simulink model "hcu_main_ADASwEPS"  (Simulink 8.2)
settings: Solver=FixedStepDiscrete  StartTime=0.0  StopTime=inf  FixedStep=0.001  RelTol=1e-3
PostLoadFcn:
  | , if any(exist('dsrtsu_mdlpostloadfcn', 'file') == [2, 3, 6]), try dsrtsu_mdlpostloadfcn('Execute', bdroot); catch fprintf('Error in PostLoadFcn (dsrtsu_mdlpostloadfcn) for model "%s":\n %s\n', bdroot, lasterr); end, end,
values from neighbouring files (symbols this model uses):
  C_TASK_1MS_S = (	C_TICK_TIME_S       )    [hcu_local_hdr.m]    (also in temp_ovrd_values.m = double(	0.001                  ))
  C_TICK_TIME_S = single(	0.005	    	)    [hcu_local_hdr.m]
  ENUM_EPSLFCSTATUS_ACTIVE = uint8(  2  )    [hcu_local_hdr.m]
  ENUM_EPSLFCSTATUS_TRANSITION = uint8(  3  )    [hcu_local_hdr.m]
  ENUM_EPSLKASTATUS_ACTIVE = uint8(  2  )    [hcu_local_hdr.m]
  ENUM_EPSMODEREQ_ANGLE = uint8(  1  )    [hcu_local_hdr.m]
  ENUM_EPSMODEREQ_INTERNAL = uint8(  0  )    [hcu_local_hdr.m]
  ENUM_EPSMODEREQ_TORQUE = uint8(  2  )    [hcu_local_hdr.m]
  ENUM_GEARPOSN_1ST = uint8(  1  )    [hcu_local_hdr.m]
  ENUM_GEARPOSN_2ND = uint8(  2  )    [hcu_local_hdr.m]
  ENUM_GEARPOSN_3RD = uint8(  3  )    [hcu_local_hdr.m]
  ENUM_GEARPOSN_4TH = uint8(  4  )    [hcu_local_hdr.m]
  ENUM_GEARPOSN_5TH = uint8(  5  )    [hcu_local_hdr.m]
  ENUM_GEARPOSN_6TH = uint8(  6  )    [hcu_local_hdr.m]
  ENUM_GEARPOSN_R = uint8(  7  )    [hcu_local_hdr.m]
  FALSE = boolean( 0 )    [hcu_local_hdr.m]
  TRUE = boolean( 1 )    [hcu_local_hdr.m]
undefined symbols (not defined in the file or in its folder): AISP_EPSCurrent_pct, AISP_TqASensorDelta_pct, AISP_TqBSensorDelta_pct, dHAL_IN, hal, INVALID_ABS1_TIMEOUT, INVALID_ABS2_TIMEOUT, INVALID_ABS3_TIMEOUT, INVALID_ABS4_TIMEOUT, INVALID_AC1_TIMEOUT, INVALID_ADASTORQ_REQ, INVALID_BCM1_TIMEOUT, INVALID_BCM2_TIMEOUT, INVALID_BOOSTER_VAC, INVALID_CSW1_TIMEOUT, INVALID_CUR_VEHDECE, INVALID_CURBRAKEDECE_REQ, INVALID_CURSTEERANG_REQ, INVALID_CURSTEERTQ_REQ, INVALID_ECM1_TIMEOUT, INVALID_ECM2_TIMEOUT, INVALID_ECM3_TIMEOUT, INVALID_ECM9_TIMEOUT, INVALID_ENG_TORQUE_FRICTIONAL, INVALID_ENG_TORQUE_INDICATED, INVALID_ENG_TORQUE_INDICATEDCOR, INVALID_ENG_TQ_MAX, INVALID_ENG_TQ_MIN, INVALID_EPAS2_TIMEOUT, INVALID_EPAS3_TIMEOUT, INVALID_EPB1_TIMEOUT, INVALID_EPS_BATTVOLT, INVALID_ESC_BATTVOLT, INVALID_GRADE, INVALID_HCU3_TIMEOUT, INVALID_HCU4_TIMEOUT, INVALID_HMI1_TIMEOUT, INVALID_HMI2_TIMEOUT, INVALID_LAT_ACC, INVALID_LONG_ACC, INVALID_MC_PRESSURE, INVALID_METER1_TIMEOUT, INVALID_METER3_TIMEOUT, INVALID_METER_VEHSPD, INVALID_ODO_METER, INVALID_OUTSIDE_TEMP, INVALID_PARKBRAKEBIND_STAT, INVALID_PEDALTQ_REQ, INVALID_SAS1_TIMEOUT, INVALID_SAS_ANGLE, INVALID_SHIFTER_POSN, INVALID_TCM1_TIMEOUT, INVALID_TCM2_TIMEOUT, INVALID_VCU1_TIMEOUT, INVALID_VCU2_TIMEOUT, INVALID_VEH_CRASH, INVALID_VEH_SPD, INVALID_WHEEL_SPD, INVALID_YAW_RATE, KHAL_MssgIdObj1_num ... (+8)
libraries: simulink x147, hcu_lib x38, rti1401lib_dio_type3 x4, rtimmsu_dsrtlib x3, app x1, rtiethernetudplib x1, rti1401lib_adc_type4 x1, rti1401lib_dac_type3 x1, inp x1, lidr x1, outp x1
(part 7 of 15)

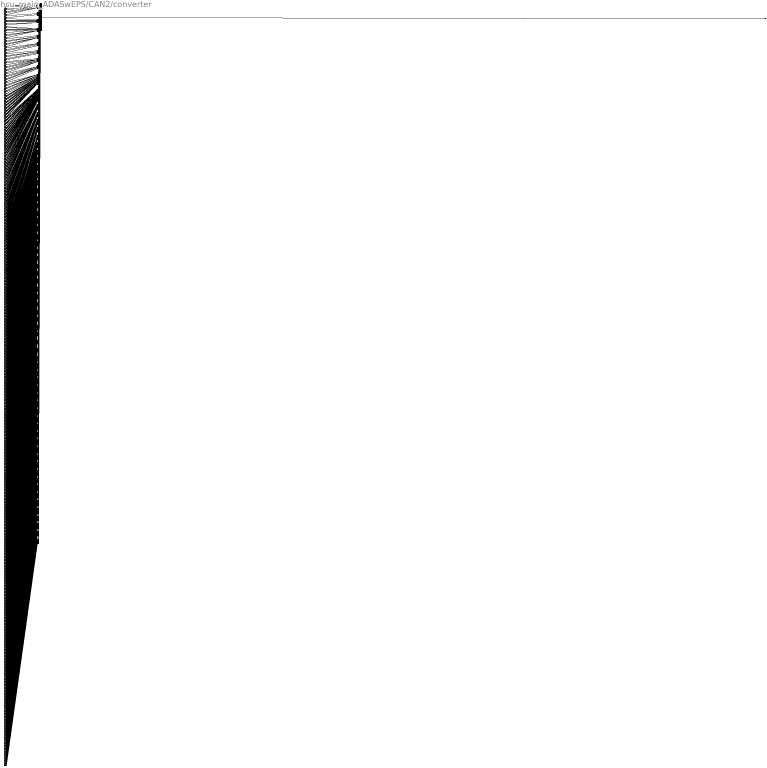
== system hcu_main_ADASwEPS/CAN2/converter ==
  in_1 : Inport
  in_2 : Inport  Port=2
  in_3 : Inport  Port=3
  in_4 : Inport  Port=4
  in_5 : Inport  Port=5
  in_6 : Inport  Port=6
  in_7 : Inport  Port=7
  in_8 : Inport  Port=8
  in_9 : Inport  Port=9
  in_10 : Inport  Port=10
  in_11 : Inport  Port=11
  in_12 : Inport  Port=12
  in_13 : Inport  Port=13
  in_14 : Inport  Port=14
  in_15 : Inport  Port=15
  in_16 : Inport  Port=16
  in_17 : Inport  Port=17
  in_18 : Inport  Port=18
  in_19 : Inport  Port=19
  in_20 : Inport  Port=20
  in_21 : Inport  Port=21
  in_22 : Inport  Port=22
  in_23 : Inport  Port=23
  in_24 : Inport  Port=24
  in_25 : Inport  Port=25
  in_26 : Inport  Port=26
  in_27 : Inport  Port=27
  in_28 : Inport  Port=28
  in_29 : Inport  Port=29
  in_30 : Inport  Port=30
  in_31 : Inport  Port=31
  in_32 : Inport  Port=32
  in_33 : Inport  Port=33
  in_34 : Inport  Port=34
  in_35 : Inport  Port=35
  in_36 : Inport  Port=36
  in_37 : Inport  Port=37
  in_38 : Inport  Port=38
  in_39 : Inport  Port=39
  in_40 : Inport  Port=40
  in_41 : Inport  Port=41
  in_42 : Inport  Port=42
  in_43 : Inport  Port=43
  in_44 : Inport  Port=44
  in_45 : Inport  Port=45
  in_46 : Inport  Port=46
  in_47 : Inport  Port=47
  in_48 : Inport  Port=48
  in_49 : Inport  Port=49
  in_50 : Inport  Port=50
  in_51 : Inport  Port=51
  in_52 : Inport  Port=52
  in_53 : Inport  Port=53
  in_54 : Inport  Port=54
  in_55 : Inport  Port=55
  in_56 : Inport  Port=56
  in_57 : Inport  Port=57
  in_58 : Inport  Port=58
  in_59 : Inport  Port=59
  in_60 : Inport  Port=60
  in_61 : Inport  Port=61
  in_62 : Inport  Port=62
  in_63 : Inport  Port=63
  in_64 : Inport  Port=64
  in_65 : Inport  Port=65
  in_66 : Inport  Port=66
  in_67 : Inport  Port=67
  in_68 : Inport  Port=68
  in_69 : Inport  Port=69
  in_70 : Inport  Port=70
  in_71 : Inport  Port=71
  in_72 : Inport  Port=72
  in_73 : Inport  Port=73
  in_74 : Inport  Port=74
  in_75 : Inport  Port=75
  in_76 : Inport  Port=76
  in_77 : Inport  Port=77
  in_78 : Inport  Port=78
  in_79 : Inport  Port=79
  in_80 : Inport  Port=80
  in_81 : Inport  Port=81
  in_82 : Inport  Port=82
  in_83 : Inport  Port=83
  in_84 : Inport  Port=84
  in_85 : Inport  Port=85
  in_86 : Inport  Port=86
  in_87 : Inport  Port=87
  in_88 : Inport  Port=88
  in_89 : Inport  Port=89
  in_90 : Inport  Port=90
  in_91 : Inport  Port=91
  in_92 : Inport  Port=92
  in_93 : Inport  Port=93
  in_94 : Inport  Port=94
  in_95 : Inport  Port=95
  in_96 : Inport  Port=96
  in_97 : Inport  Port=97
  in_98 : Inport  Port=98
  in_99 : Inport  Port=99
  in_100 : Inport  Port=100
  in_101 : Inport  Port=101
  in_102 : Inport  Port=102
  in_103 : Inport  Port=103
  in_104 : Inport  Port=104
  in_105 : Inport  Port=105
  in_106 : Inport  Port=106
  in_107 : Inport  Port=107
  in_108 : Inport  Port=108
  in_109 : Inport  Port=109
  in_110 : Inport  Port=110
  in_111 : Inport  Port=111
  in_112 : Inport  Port=112
  in_113 : Inport  Port=113
  in_114 : Inport  Port=114
  in_115 : Inport  Port=115
  in_116 : Inport  Port=116
  in_117 : Inport  Port=117
  in_118 : Inport  Port=118
  in_119 : Inport  Port=119
  in_120 : Inport  Port=120
  in_121 : Inport  Port=121
  in_122 : Inport  Port=122
  in_123 : Inport  Port=123
  in_124 : Inport  Port=124
  in_125 : Inport  Port=125
  in_126 : Inport  Port=126
  in_127 : Inport  Port=127
  in_128 : Inport  Port=128
  in_129 : Inport  Port=129
  in_130 : Inport  Port=130
  in_131 : Inport  Port=131
  in_132 : Inport  Port=132
  in_133 : Inport  Port=133
  in_134 : Inport  Port=134
  in_135 : Inport  Port=135
  in_136 : Inport  Port=136
  in_137 : Inport  Port=137
  in_138 : Inport  Port=138
  in_139 : Inport  Port=139
  in_140 : Inport  Port=140
  in_141 : Inport  Port=141
  in_142 : Inport  Port=142
  in_143 : Inport  Port=143
  in_144 : Inport  Port=144
  in_145 : Inport  Port=145
  in_146 : Inport  Port=146
  in_147 : Inport  Port=147
  in_148 : Inport  Port=148
  in_149 : Inport  Port=149
  in_150 : Inport  Port=150
  in_151 : Inport  Port=151
  in_152 : Inport  Port=152
  in_153 : Inport  Port=153
  in_154 : Inport  Port=154
  in_155 : Inport  Port=155
  in_156 : Inport  Port=156
  in_157 : Inport  Port=157
  in_158 : Inport  Port=158
  in_159 : Inport  Port=159
  in_160 : Inport  Port=160
  in_161 : Inport  Port=161
  in_162 : Inport  Port=162
  in_163 : Inport  Port=163
  in_164 : Inport  Port=164
  in_165 : Inport  Port=165
  in_166 : Inport  Port=166
  in_167 : Inport  Port=167
  in_168 : Inport  Port=168
  in_169 : Inport  Port=169
  in_170 : Inport  Port=170
  in_171 : Inport  Port=171
  in_172 : Inport  Port=172
  in_173 : Inport  Port=173
  in_174 : Inport  Port=174
  in_175 : Inport  Port=175
  in_176 : Inport  Port=176
  in_177 : Inport  Port=177
  in_178 : Inport  Port=178
  in_179 : Inport  Port=179
  in_180 : Inport  Port=180
  in_181 : Inport  Port=181
  in_182 : Inport  Port=182
  in_183 : Inport  Port=183
  in_184 : Inport  Port=184
  in_185 : Inport  Port=185
  in_186 : Inport  Port=186
  in_187 : Inport  Port=187
  in_188 : Inport  Port=188
  in_189 : Inport  Port=189
  in_190 : Inport  Port=190
  in_191 : Inport  Port=191
  in_192 : Inport  Port=192
  in_193 : Inport  Port=193
  in_194 : Inport  Port=194
  in_195 : Inport  Port=195
  in_196 : Inport  Port=196
  in_197 : Inport  Port=197
  in_198 : Inport  Port=198
  in_199 : Inport  Port=199
  in_200 : Inport  Port=200
  in_201 : Inport  Port=201
  in_202 : Inport  Port=202
  in_203 : Inport  Port=203
  in_204 : Inport  Port=204
  in_205 : Inport  Port=205
  in_206 : Inport  Port=206
  in_207 : Inport  Port=207
  in_208 : Inport  Port=208
  in_209 : Inport  Port=209
  in_210 : Inport  Port=210
  in_211 : Inport  Port=211
  in_212 : Inport  Port=212
  in_213 : Inport  Port=213
  in_214 : Inport  Port=214
  in_215 : Inport  Port=215
  in_216 : Inport  Port=216
  in_217 : Inport  Port=217
  in_218 : Inport  Port=218
  in_219 : Inport  Port=219
  in_220 : Inport  Port=220
  in_221 : Inport  Port=221
  in_222 : Inport  Port=222
  in_223 : Inport  Port=223
  in_224 : Inport  Port=224
  in_225 : Inport  Port=225
  in_226 : Inport  Port=226
  in_227 : Inport  Port=227
  in_228 : Inport  Port=228
  in_229 : Inport  Port=229
  in_230 : Inport  Port=230
  in_231 : Inport  Port=231
  in_232 : Inport  Port=232
  in_233 : Inport  Port=233
  in_234 : Inport  Port=234
  in_235 : Inport  Port=235
  in_236 : Inport  Port=236
  in_237 : Inport  Port=237
  in_238 : Inport  Port=238
  in_239 : Inport  Port=239
  in_240 : Inport  Port=240
  in_241 : Inport  Port=241
  in_242 : Inport  Port=242
  in_243 : Inport  Port=243
  in_244 : Inport  Port=244
  in_245 : Inport  Port=245
  in_246 : Inport  Port=246
  in_247 : Inport  Port=247
  in_248 : Inport  Port=248
  in_249 : Inport  Port=249
  in_250 : Inport  Port=250
  in_251 : Inport  Port=251
  in_252 : Inport  Port=252
  in_253 : Inport  Port=253
  in_254 : Inport  Port=254
  in_255 : Inport  Port=255
  in_256 : Inport  Port=256
  in_257 : Inport  Port=257
  in_258 : Inport  Port=258
  in_259 : Inport  Port=259
  in_260 : Inport  Port=260
  in_261 : Inport  Port=261
  in_262 : Inport  Port=262
  in_263 : Inport  Port=263
  in_264 : Inport  Port=264
  in_265 : Inport  Port=265
  in_266 : Inport  Port=266
  in_267 : Inport  Port=267
  in_268 : Inport  Port=268
  in_269 : Inport  Port=269
  in_270 : Inport  Port=270
  in_271 : Inport  Port=271
  in_272 : Inport  Port=272
  in_273 : Inport  Port=273
  in_274 : Inport  Port=274
  in_275 : Inport  Port=275
  in_276 : Inport  Port=276
  in_277 : Inport  Port=277
  in_278 : Inport  Port=278
  in_279 : Inport  Port=279
  in_280 : Inport  Port=280
  in_281 : Inport  Port=281
  in_282 : Inport  Port=282
  in_283 : Inport  Port=283
  in_284 : Inport  Port=284
  in_285 : Inport  Port=285
  in_286 : Inport  Port=286
  in_287 : Inport  Port=287
  in_288 : Inport  Port=288
  in_289 : Inport  Port=289
  in_290 : Inport  Port=290
  in_291 : Inport  Port=291
  in_292 : Inport  Port=292
  in_293 : Inport  Port=293
  in_294 : Inport  Port=294
  in_295 : Inport  Port=295
  in_296 : Inport  Port=296
  in_297 : Inport  Port=297
  in_298 : Inport  Port=298
  in_299 : Inport  Port=299
  in_300 : Inport  Port=300
  in_301 : Inport  Port=301
  in_302 : Inport  Port=302
  in_303 : Inport  Port=303
  in_304 : Inport  Port=304
  in_305 : Inport  Port=305
  in_306 : Inport  Port=306
  in_307 : Inport  Port=307
  in_308 : Inport  Port=308
  in_309 : Inport  Port=309
  in_310 : Inport  Port=310
  in_311 : Inport  Port=311
  in_312 : Inport  Port=312
  in_313 : Inport  Port=313
  in_314 : Inport  Port=314
  in_315 : Inport  Port=315
  in_316 : Inport  Port=316
  in_317 : Inport  Port=317
  in_318 : Inport  Port=318
  in_319 : Inport  Port=319
  in_320 : Inport  Port=320
  in_321 : Inport  Port=321
  in_322 : Inport  Port=322
  in_323 : Inport  Port=323
  in_324 : Inport  Port=324
  in_325 : Inport  Port=325
  in_326 : Inport  Port=326
  in_327 : Inport  Port=327
  in_328 : Inport  Port=328
  in_329 : Inport  Port=329
  in_330 : Inport  Port=330
  in_331 : Inport  Port=331
  in_332 : Inport  Port=332
  in_333 : Inport  Port=333
  in_334 : Inport  Port=334
  in_335 : Inport  Port=335
  in_336 : Inport  Port=336
  in_337 : Inport  Port=337
  in_338 : Inport  Port=338
  in_339 : Inport  Port=339
  in_340 : Inport  Port=340
  in_341 : Inport  Port=341
  in_342 : Inport  Port=342
  in_343 : Inport  Port=343
  in_344 : Inport  Port=344
  in_345 : Inport  Port=345
  in_346 : Inport  Port=346
  in_347 : Inport  Port=347
  in_348 : Inport  Port=348
  in_349 : Inport  Port=349
  in_350 : Inport  Port=350
  in_351 : Inport  Port=351
  in_352 : Inport  Port=352
  in_353 : Inport  Port=353
  in_354 : Inport  Port=354
  in_355 : Inport  Port=355
  in_356 : Inport  Port=356
  in_357 : Inport  Port=357
  in_358 : Inport  Port=358
  in_359 : Inport  Port=359
  in_360 : Inport  Port=360
  in_361 : Inport  Port=361
  in_362 : Inport  Port=362
  in_363 : Inport  Port=363
  in_364 : Inport  Port=364
  in_365 : Inport  Port=365
  in_366 : Inport  Port=366
  in_367 : Inport  Port=367
  in_368 : Inport  Port=368
  in_369 : Inport  Port=369
  in_370 : Inport  Port=370
  in_371 : Inport  Port=371
  in_372 : Inport  Port=372
  in_373 : Inport  Port=373
  in_374 : Inport  Port=374
  in_375 : Inport  Port=375
  in_376 : Inport  Port=376
  in_377 : Inport  Port=377
  in_378 : Inport  Port=378
  in_379 : Inport  Port=379
  in_380 : Inport  Port=380
  in_381 : Inport  Port=381
  in_382 : Inport  Port=382
  in_383 : Inport  Port=383
  in_384 : Inport  Port=384
  in_385 : Inport  Port=385
  in_386 : Inport  Port=386
  in_387 : Inport  Port=387
  in_388 : Inport  Port=388
  in_389 : Inport  Port=389
  in_390 : Inport  Port=390
  in_391 : Inport  Port=391
  in_392 : Inport  Port=392
  in_393 : Inport  Port=393
  in_394 : Inport  Port=394
  in_395 : Inport  Port=395
  in_396 : Inport  Port=396
  in_397 : Inport  Port=397
  in_398 : Inport  Port=398
  in_399 : Inport  Port=399
  in_400 : Inport  Port=400
  in_401 : Inport  Port=401
  in_402 : Inport  Port=402
  in_403 : Inport  Port=403
  in_404 : Inport  Port=404
  in_405 : Inport  Port=405
  in_406 : Inport  Port=406
  in_407 : Inport  Port=407
  in_408 : Inport  Port=408
  in_409 : Inport  Port=409
  in_410 : Inport  Port=410
  in_411 : Inport  Port=411
  in_412 : Inport  Port=412
  in_413 : Inport  Port=413
  in_414 : Inport  Port=414
  in_415 : Inport  Port=415
  in_416 : Inport  Port=416
  in_417 : Inport  Port=417
  in_418 : Inport  Port=418
  in_419 : Inport  Port=419
  in_420 : Inport  Port=420
  in_421 : Inport  Port=421
  in_422 : Inport  Port=422
  in_423 : Inport  Port=423
  in_424 : Inport  Port=424
  in_425 : Inport  Port=425
  in_426 : Inport  Port=426
  in_427 : Inport  Port=427
  in_428 : Inport  Port=428
  in_429 : Inport  Port=429
  in_430 : Inport  Port=430
  in_431 : Inport  Port=431
  in_432 : Inport  Port=432
  in_433 : Inport  Port=433
  in_434 : Inport  Port=434
  in_435 : Inport  Port=435
  in_436 : Inport  Port=436
  in_437 : Inport  Port=437
  in_438 : Inport  Port=438
  in_439 : Inport  Port=439
  in_440 : Inport  Port=440
  in_441 : Inport  Port=441
  in_442 : Inport  Port=442
  in_443 : Inport  Port=443
  in_444 : Inport  Port=444
  in_445 : Inport  Port=445
  in_446 : Inport  Port=446
  in_447 : Inport  Port=447
  in_448 : Inport  Port=448
  in_449 : Inport  Port=449
  in_450 : Inport  Port=450
  in_451 : Inport  Port=451
  in_452 : Inport  Port=452
  in_453 : Inport  Port=453
  in_454 : Inport  Port=454
  in_455 : Inport  Port=455
  in_456 : Inport  Port=456
  in_457 : Inport  Port=457
  in_458 : Inport  Port=458
  in_459 : Inport  Port=459
  in_460 : Inport  Port=460
  in_461 : Inport  Port=461
  in_462 : Inport  Port=462
  in_463 : Inport  Port=463
  in_464 : Inport  Port=464
  in_465 : Inport  Port=465
  in_466 : Inport  Port=466
  in_467 : Inport  Port=467
  in_468 : Inport  Port=468
  in_469 : Inport  Port=469
  in_470 : Inport  Port=470
  in_471 : Inport  Port=471
  in_472 : Inport  Port=472
  in_473 : Inport  Port=473
  in_474 : Inport  Port=474
  in_475 : Inport  Port=475
  in_476 : Inport  Port=476
  in_477 : Inport  Port=477
  in_478 : Inport  Port=478
  in_479 : Inport  Port=479
  in_480 : Inport  Port=480
  in_481 : Inport  Port=481
  in_482 : Inport  Port=482
  in_483 : Inport  Port=483
  in_484 : Inport  Port=484
  in_485 : Inport  Port=485
  in_486 : Inport  Port=486
  in_487 : Inport  Port=487
  in_488 : Inport  Port=488
  in_489 : Inport  Port=489
  in_490 : Inport  Port=490
  in_491 : Inport  Port=491
  in_492 : Inport  Port=492
  in_493 : Inport  Port=493
  in_494 : Inport  Port=494
  in_495 : Inport  Port=495
  in_496 : Inport  Port=496
  in_497 : Inport  Port=497
  in_498 : Inport  Port=498
  in_499 : Inport  Port=499
  in_500 : Inport  Port=500
  in_501 : Inport  Port=501
  in_502 : Inport  Port=502
  in_503 : Inport  Port=503
  in_504 : Inport  Port=504
  in_505 : Inport  Port=505
  in_506 : Inport  Port=506
  in_507 : Inport  Port=507
  in_508 : Inport  Port=508
  in_509 : Inport  Port=509
  in_510 : Inport  Port=510
  in_511 : Inport  Port=511
  in_512 : Inport  Port=512
  in_513 : Inport  Port=513
  in_514 : Inport  Port=514
  in_515 : Inport  Port=515
  in_516 : Inport  Port=516
  in_517 : Inport  Port=517
  in_518 : Inport  Port=518
  in_519 : Inport  Port=519
  in_520 : Inport  Port=520
  in_521 : Inport  Port=521
  in_522 : Inport  Port=522
  in_523 : Inport  Port=523
  in_524 : Inport  Port=524
  in_525 : Inport  Port=525
  in_526 : Inport  Port=526
  in_527 : Inport  Port=527
  in_528 : Inport  Port=528
  in_529 : Inport  Port=529
  in_530 : Inport  Port=530
  in_531 : Inport  Port=531
  in_532 : Inport  Port=532
  in_533 : Inport  Port=533
  in_534 : Inport  Port=534
  in_535 : Inport  Port=535
  in_536 : Inport  Port=536
  in_537 : Inport  Port=537
  in_538 : Inport  Port=538
  in_539 : Inport  Port=539
  in_540 : Inport  Port=540
  in_541 : Inport  Port=541
  in_542 : Inport  Port=542
  in_543 : Inport  Port=543
  in_544 : Inport  Port=544
  in_545 : Inport  Port=545
  in_546 : Inport  Port=546
  in_547 : Inport  Port=547
  in_548 : Inport  Port=548
  in_549 : Inport  Port=549
  in_550 : Inport  Port=550
  in_551 : Inport  Port=551
  in_552 : Inport  Port=552
  in_553 : Inport  Port=553
  in_554 : Inport  Port=554
  in_555 : Inport  Port=555
  in_556 : Inport  Port=556
  in_557 : Inport  Port=557
  in_558 : Inport  Port=558
  in_559 : Inport  Port=559
  in_560 : Inport  Port=560
  in_561 : Inport  Port=561
  in_562 : Inport  Port=562
  in_563 : Inport  Port=563
  in_564 : Inport  Port=564
  in_565 : Inport  Port=565
  in_566 : Inport  Port=566
  in_567 : Inport  Port=567
  in_568 : Inport  Port=568
  in_569 : Inport  Port=569
  in_570 : Inport  Port=570
  in_571 : Inport  Port=571
  in_572 : Inport  Port=572
  in_573 : Inport  Port=573
  in_574 : Inport  Port=574
  in_575 : Inport  Port=575
  in_576 : Inport  Port=576
  in_577 : Inport  Port=577
  in_578 : Inport  Port=578
  in_579 : Inport  Port=579
  in_580 : Inport  Port=580
  in_581 : Inport  Port=581
  in_582 : Inport  Port=582
  in_583 : Inport  Port=583
  in_584 : Inport  Port=584
  in_585 : Inport  Port=585
  in_586 : Inport  Port=586
  in_587 : Inport  Port=587
  in_588 : Inport  Port=588
  in_589 : Inport  Port=589
  in_590 : Inport  Port=590
  in_591 : Inport  Port=591
  in_592 : Inport  Port=592
  in_593 : Inport  Port=593
  in_594 : Inport  Port=594
  in_595 : Inport  Port=595
  in_596 : Inport  Port=596
  in_597 : Inport  Port=597
  in_598 : Inport  Port=598
  in_599 : Inport  Port=599
  in_600 : Inport  Port=600
  in_601 : Inport  Port=601
  in_602 : Inport  Port=602
  in_603 : Inport  Port=603
  in_604 : Inport  Port=604
  in_605 : Inport  Port=605
  in_606 : Inport  Port=606
  in_607 : Inport  Port=607
  in_608 : Inport  Port=608
  in_609 : Inport  Port=609
  in_610 : Inport  Port=610
  in_611 : Inport  Port=611
  in_612 : Inport  Port=612
  in_613 : Inport  Port=613
  in_614 : Inport  Port=614
  in_615 : Inport  Port=615
  in_616 : Inport  Port=616
  in_617 : Inport  Port=617
  in_618 : Inport  Port=618
  in_619 : Inport  Port=619
  in_620 : Inport  Port=620
  in_621 : Inport  Port=621
  in_622 : Inport  Port=622
  in_623 : Inport  Port=623
  in_624 : Inport  Port=624
  in_625 : Inport  Port=625
  in_626 : Inport  Port=626
  in_627 : Inport  Port=627
  in_628 : Inport  Port=628
  in_629 : Inport  Port=629
  in_630 : Inport  Port=630
  in_631 : Inport  Port=631
  in_632 : Inport  Port=632
  in_633 : Inport  Port=633
  in_634 : Inport  Port=634
  in_635 : Inport  Port=635
  in_636 : Inport  Port=636
  in_637 : Inport  Port=637
  in_638 : Inport  Port=638
  in_639 : Inport  Port=639
  in_640 : Inport  Port=640
  in_641 : Inport  Port=641
  in_642 : Inport  Port=642
  in_643 : Inport  Port=643
  in_644 : Inport  Port=644
  in_645 : Inport  Port=645
  in_646 : Inport  Port=646
  in_647 : Inport  Port=647
  in_648 : Inport  Port=648
  in_649 : Inport  Port=649
  in_650 : Inport  Port=650
  in_651 : Inport  Port=651
  in_652 : Inport  Port=652
  in_653 : Inport  Port=653
  in_654 : Inport  Port=654
  in_655 : Inport  Port=655
  in_656 : Inport  Port=656
  in_657 : Inport  Port=657
  in_658 : Inport  Port=658
  in_659 : Inport  Port=659
  in_660 : Inport  Port=660
  in_661 : Inport  Port=661
  in_662 : Inport  Port=662
  in_663 : Inport  Port=663
  in_664 : Inport  Port=664
  in_665 : Inport  Port=665
  in_666 : Inport  Port=666
  in_667 : Inport  Port=667
  in_668 : Inport  Port=668
  in_669 : Inport  Port=669
  in_670 : Inport  Port=670
  in_671 : Inport  Port=671
  in_672 : Inport  Port=672
  in_673 : Inport  Port=673
  in_674 : Inport  Port=674
  in_675 : Inport  Port=675
  in_676 : Inport  Port=676
  in_677 : Inport  Port=677
  in_678 : Inport  Port=678
  in_679 : Inport  Port=679
  in_680 : Inport  Port=680
  in_681 : Inport  Port=681
  in_682 : Inport  Port=682
  in_683 : Inport  Port=683
  in_684 : Inport  Port=684
  in_685 : Inport  Port=685
  in_686 : Inport  Port=686
  in_687 : Inport  Port=687
  in_688 : Inport  Port=688
  in_689 : Inport  Port=689
  in_690 : Inport  Port=690
  in_691 : Inport  Port=691
  in_692 : Inport  Port=692
  in_693 : Inport  Port=693
  in_694 : Inport  Port=694
  in_695 : Inport  Port=695
  in_696 : Inport  Port=696
  in_697 : Inport  Port=697
  in_698 : Inport  Port=698
  in_699 : Inport  Port=699
  in_700 : Inport  Port=700
  in_701 : Inport  Port=701
  in_702 : Inport  Port=702
  in_703 : Inport  Port=703
  in_704 : Inport  Port=704
  in_705 : Inport  Port=705
  in_706 : Inport  Port=706
  in_707 : Inport  Port=707
  in_708 : Inport  Port=708
  in_709 : Inport  Port=709
  in_710 : Inport  Port=710
  in_711 : Inport  Port=711
  in_712 : Inport  Port=712
  in_713 : Inport  Port=713
  in_714 : Inport  Port=714
  in_715 : Inport  Port=715
  in_716 : Inport  Port=716
  in_717 : Inport  Port=717
  in_718 : Inport  Port=718
  in_719 : Inport  Port=719
  in_720 : Inport  Port=720
  in_721 : Inport  Port=721
  in_722 : Inport  Port=722
  in_723 : Inport  Port=723
  in_724 : Inport  Port=724
  in_725 : Inport  Port=725
  in_726 : Inport  Port=726
  in_727 : Inport  Port=727
  in_728 : Inport  Port=728
  in_729 : Inport  Port=729
  in_730 : Inport  Port=730
  in_731 : Inport  Port=731
  in_732 : Inport  Port=732
  in_733 : Inport  Port=733
  in_734 : Inport  Port=734
  in_735 : Inport  Port=735
  in_736 : Inport  Port=736
  in_737 : Inport  Port=737
  in_738 : Inport  Port=738
  in_739 : Inport  Port=739
  in_740 : Inport  Port=740
  in_741 : Inport  Port=741
  in_742 : Inport  Port=742
  in_743 : Inport  Port=743
  in_744 : Inport  Port=744
  in_745 : Inport  Port=745
  in_746 : Inport  Port=746
  in_747 : Inport  Port=747
  in_748 : Inport  Port=748
  in_749 : Inport  Port=749
  in_750 : Inport  Port=750
  in_751 : Inport  Port=751
  in_752 : Inport  Port=752
  in_753 : Inport  Port=753
  in_754 : Inport  Port=754
  in_755 : Inport  Port=755
  in_756 : Inport  Port=756
  in_757 : Inport  Port=757
  in_758 : Inport  Port=758
  in_759 : Inport  Port=759
  in_760 : Inport  Port=760
  in_761 : Inport  Port=761
  in_762 : Inport  Port=762
  in_763 : Inport  Port=763
  in_764 : Inport  Port=764
  in_765 : Inport  Port=765
  in_766 : Inport  Port=766
  in_767 : Inport  Port=767
  in_768 : Inport  Port=768
  in_769 : Inport  Port=769
  in_770 : Inport  Port=770
  in_771 : Inport  Port=771
  in_772 : Inport  Port=772
  IBEO1 : BusCreator  Inputs=7
  IBEO2 : BusCreator  Inputs=2
  IBEO3 : BusCreator  Inputs=5
  IBEO4 : BusCreator  Inputs=8
  IBEO5 : BusCreator  Inputs=6
  IBEO6 : BusCreator
  IBEO7 : BusCreator  Inputs=5
  IBEO8 : BusCreator  Inputs=8
  LKA_Left_Lane_A : BusCreator  Inputs=6
  LKA_Left_Lane_B : BusCreator  Inputs=17
  LKA_Right_Lane_A : BusCreator  Inputs=6
  LKA_Right_Lane_B : BusCreator  Inputs=17
  Mux : BusCreator  Inputs=71
  ObstacleDataA{1..10} (10 alike) : BusCreator  Inputs=13
  ObstacleDataB{1..10} (10 alike) : BusCreator  Inputs=12
  ObstacleDataC{1..10} (10 alike) : BusCreator  Inputs=8
  ObstacleStatusA : BusCreator  Inputs=11
  ObstacleStatusB : BusCreator  Inputs=2
  ObstacleStatusC : BusCreator
  RTICANMMCaptureMessage_{1..25} (25 alike) : BusCreator  Inputs=13
  Road_Information : BusCreator  Inputs=9
  out : Outport
  wires:
  in_1/1 -> IBEO1/1  "HeaderCounter"
  IBEO1/1 -> Mux/1  "IBEO1"
  in_2/1 -> IBEO1/2  "ObjDataInfoFlag_vel"
  in_3/1 -> IBEO1/3  "ObjDataInfoFlag_box"
  in_4/1 -> IBEO1/4  "SensorTemp"
  in_5/1 -> IBEO1/5  "SensorViewRange"
  in_6/1 -> IBEO1/6  "NumberOfObject"
  in_7/1 -> IBEO1/7  "Version"
  in_8/1 -> IBEO2/1  "NTP_fractional_seconds"
  IBEO2/1 -> Mux/2  "IBEO2"
  in_9/1 -> IBEO2/2  "NTP_seconds"
  in_10/1 -> IBEO3/1  "VelocityY"
  IBEO3/1 -> Mux/3  "IBEO3"
  in_11/1 -> IBEO3/2  "VelocityX"
  in_12/1 -> IBEO3/3  "PositionY"
  in_13/1 -> IBEO3/4  "PositionX"
  in_14/1 -> IBEO3/5  "ObjID"
  in_15/1 -> IBEO4/1  "VelocityYSigma"
  IBEO4/1 -> Mux/4  "IBEO4"
  in_16/1 -> IBEO4/2  "VelocityXSigma"
  in_17/1 -> IBEO4/3  "PositionYSigma"
  in_18/1 -> IBEO4/4  "PositionXSigma"
  in_19/1 -> IBEO4/5  "ObjTimeOffset"
  in_20/1 -> IBEO4/6  "ObjPredictionAge"
  in_21/1 -> IBEO4/7  "ObjAge"
  in_22/1 -> IBEO4/8  "ObjID"
  in_23/1 -> IBEO5/1  "BoxCenterY"
  IBEO5/1 -> Mux/5  "IBEO5"
  in_24/1 -> IBEO5/2  "BoxCenterX"
  in_25/1 -> IBEO5/3  "ObjClassAge"
  in_26/1 -> IBEO5/4  "ObjClassCertainty"
  in_27/1 -> IBEO5/5  "ObjClassification"
  in_28/1 -> IBEO5/6  "ObjID"
  in_29/1 -> IBEO6/1  "BoxOrientation"
  IBEO6/1 -> Mux/6  "IBEO6"
  in_30/1 -> IBEO6/2  "BoxSizeY"
  in_31/1 -> IBEO6/3  "BoxSizeX"
  in_32/1 -> IBEO6/4  "ObjID"
  in_33/1 -> IBEO7/1  "StartPointY"
  IBEO7/1 -> Mux/7  "IBEO7"
  in_34/1 -> IBEO7/2  "StartPointX"
  in_35/1 -> IBEO7/3  "ClosestContourPointNum"
  in_36/1 -> IBEO7/4  "NumberOfContourPoints"
  in_37/1 -> IBEO7/5  "ObjID"
  in_38/1 -> IBEO8/1  "yOffset3"
  IBEO8/1 -> Mux/8  "IBEO8"
  in_39/1 -> IBEO8/2  "xOffset3"
  in_40/1 -> IBEO8/3  "yOffset2"
  in_41/1 -> IBEO8/4  "xOffset2"
  in_42/1 -> IBEO8/5  "yOffset"
  in_43/1 -> IBEO8/6  "xOffset"
  in_44/1 -> IBEO8/7  "ContourMessageNum"
  in_45/1 -> IBEO8/8  "ObjID"
  in_46/1 -> LKA_Left_Lane_A/1  "Lane_Type"
  LKA_Left_Lane_A/1 -> Mux/9  "LKA_Left_Lane_A"
  in_47/1 -> LKA_Left_Lane_A/2  "Quality"
  in_48/1 -> LKA_Left_Lane_A/3  "Position"
  in_49/1 -> LKA_Left_Lane_A/4  "Curvature"
  in_50/1 -> LKA_Left_Lane_A/5  "Curvature_Derivative"
  in_51/1 -> LKA_Left_Lane_A/6  "Width_left_marking"
  in_52/1 -> LKA_Left_Lane_B/1  "Heading_Angle"
  LKA_Left_Lane_B/1 -> Mux/10  "LKA_Left_Lane_B"
  in_53/1 -> LKA_Left_Lane_B/2  "View_Range_Start"
  in_54/1 -> LKA_Left_Lane_B/3  "View_Range_End"
  in_55/1 -> LKA_Left_Lane_B/4  "Lane_Crossing"
  in_56/1 -> LKA_Left_Lane_B/5  "Lane_mark_color"
  in_57/1 -> LKA_Left_Lane_B/6  "PRED_DIST_BASED_EXTRAPOLATION"
  in_58/1 -> LKA_Left_Lane_B/7  "PRED_OTHER_SIDE"
  in_59/1 -> LKA_Left_Lane_B/8  "PRED_OVERRIDE"
  in_60/1 -> LKA_Left_Lane_B/9  "PRED_OCCLUDED_LM_EXTRAPOLATION"
  in_61/1 -> LKA_Left_Lane_B/10  "PRED_HEADWAY_ORIENTED"
  in_62/1 -> LKA_Left_Lane_B/11  "Reserved1_laneB"
  in_63/1 -> LKA_Left_Lane_B/12  "PRED_SOURCE_DIVERGING_LANES"
  in_64/1 -> LKA_Left_Lane_B/13  "PRED_SOURCE_GUARDRAIL_SHADOW"
  in_65/1 -> LKA_Left_Lane_B/14  "PRED_SOURCE_HWE_SPAIN"
  in_66/1 -> LKA_Left_Lane_B/15  "PRED_SOURCE_STD"
  in_67/1 -> LKA_Left_Lane_B/16  "PRED_SOURCE_VRTL_MERGE"
  in_68/1 -> LKA_Left_Lane_B/17  "TLC"
  in_69/1 -> LKA_Right_Lane_A/1  "Lane_Type"
  LKA_Right_Lane_A/1 -> Mux/11  "LKA_Right_Lane_A"
  in_70/1 -> LKA_Right_Lane_A/2  "Quality"
  in_71/1 -> LKA_Right_Lane_A/3  "Position"
  in_72/1 -> LKA_Right_Lane_A/4  "Curvature"
  in_73/1 -> LKA_Right_Lane_A/5  "Curvature_Derivative"
  in_74/1 -> LKA_Right_Lane_A/6  "Width_right_marking"
  in_75/1 -> LKA_Right_Lane_B/1  "Heading_Angle"
  LKA_Right_Lane_B/1 -> Mux/12  "LKA_Right_Lane_B"
  in_76/1 -> LKA_Right_Lane_B/2  "View_Range_Start"
  in_77/1 -> LKA_Right_Lane_B/3  "View_Range_End"
  in_78/1 -> LKA_Right_Lane_B/4  "Lane_Crossing"
  in_79/1 -> LKA_Right_Lane_B/5  "Lane_mark_color"
  in_80/1 -> LKA_Right_Lane_B/6  "PRED_DIST_BASED_EXTRAPOLATION"
  in_81/1 -> LKA_Right_Lane_B/7  "PRED_OTHER_SIDE"
  in_82/1 -> LKA_Right_Lane_B/8  "PRED_OVERRIDE"
  in_83/1 -> LKA_Right_Lane_B/9  "PRED_OCCLUDED_LM_EXTRAPOLATION"
  in_84/1 -> LKA_Right_Lane_B/10  "PRED_HEADWAY_ORIENTED"
  in_85/1 -> LKA_Right_Lane_B/11  "Reserved1_laneB"
  in_86/1 -> LKA_Right_Lane_B/12  "PRED_SOURCE_DIVERGING_LANES"
  in_87/1 -> LKA_Right_Lane_B/13  "PRED_SOURCE_GUARDRAIL_SHADOW"
  in_88/1 -> LKA_Right_Lane_B/14  "PRED_SOURCE_HWE_SPAIN"
  in_89/1 -> LKA_Right_Lane_B/15  "PRED_SOURCE_STD"
  in_90/1 -> LKA_Right_Lane_B/16  "PRED_SOURCE_VRTL_MERGE"
  in_91/1 -> LKA_Right_Lane_B/17  "TLC"
  in_92/1 -> ObstacleDataA1/1  "ObstacleID"
  ObstacleDataA1/1 -> Mux/13  "ObstacleDataA1"
  in_93/1 -> ObstacleDataA1/2  "ObstaclePosX"
  in_94/1 -> ObstacleDataA1/3  "reserved_4"
  in_95/1 -> ObstacleDataA1/4  "ObstaclePosY"
  in_96/1 -> ObstacleDataA1/5  "BlinkerInfo"
  in_97/1 -> ObstacleDataA1/6  "Move_in_and_Out"
  in_98/1 -> ObstacleDataA1/7  "ObstacleVelX"
  in_99/1 -> ObstacleDataA1/8  "ObstacleType"
  in_100/1 -> ObstacleDataA1/9  "reserved_1"
  in_101/1 -> ObstacleDataA1/10  "ObstacleStatus"
  in_102/1 -> ObstacleDataA1/11  "ObstacleBrakeLights"
  in_103/1 -> ObstacleDataA1/12  "reserved_2"
  in_104/1 -> ObstacleDataA1/13  "ObstacleValid"
  in_105/1 -> ObstacleDataA10/1  "ObstacleID"
  ObstacleDataA10/1 -> Mux/14  "ObstacleDataA10"
  in_106/1 -> ObstacleDataA10/2  "ObstaclePosX"
  in_107/1 -> ObstacleDataA10/3  "reserved_4"
  in_108/1 -> ObstacleDataA10/4  "ObstaclePosY"
  in_109/1 -> ObstacleDataA10/5  "BlinkerInfo"
  in_110/1 -> ObstacleDataA10/6  "Move_in_and_Out"
  in_111/1 -> ObstacleDataA10/7  "ObstacleVelX"
  in_112/1 -> ObstacleDataA10/8  "ObstacleType"
  in_113/1 -> ObstacleDataA10/9  "reserved_1"
  in_114/1 -> ObstacleDataA10/10  "ObstacleStatus"
  in_115/1 -> ObstacleDataA10/11  "ObstacleBrakeLights"
  in_116/1 -> ObstacleDataA10/12  "reserved_2"
  in_117/1 -> ObstacleDataA10/13  "ObstacleValid"
  in_118/1 -> ObstacleDataA2/1  "ObstacleID"
  ObstacleDataA2/1 -> Mux/15  "ObstacleDataA2"
  in_119/1 -> ObstacleDataA2/2  "ObstaclePosX"
  in_120/1 -> ObstacleDataA2/3  "reserved_4"
  in_121/1 -> ObstacleDataA2/4  "ObstaclePosY"
  in_122/1 -> ObstacleDataA2/5  "BlinkerInfo"
  in_123/1 -> ObstacleDataA2/6  "Move_in_and_Out"
  in_124/1 -> ObstacleDataA2/7  "ObstacleVelX"
  in_125/1 -> ObstacleDataA2/8  "ObstacleType"
  in_126/1 -> ObstacleDataA2/9  "reserved_1"
  in_127/1 -> ObstacleDataA2/10  "ObstacleStatus"
  in_128/1 -> ObstacleDataA2/11  "ObstacleBrakeLights"
  in_129/1 -> ObstacleDataA2/12  "reserved_2"
  in_130/1 -> ObstacleDataA2/13  "ObstacleValid"
  in_131/1 -> ObstacleDataA3/1  "ObstacleID"
  ObstacleDataA3/1 -> Mux/16  "ObstacleDataA3"
  in_132/1 -> ObstacleDataA3/2  "ObstaclePosX"
  in_133/1 -> ObstacleDataA3/3  "reserved_4"
  in_134/1 -> ObstacleDataA3/4  "ObstaclePosY"
  in_135/1 -> ObstacleDataA3/5  "BlinkerInfo"
  in_136/1 -> ObstacleDataA3/6  "Move_in_and_Out"
  in_137/1 -> ObstacleDataA3/7  "ObstacleVelX"
  in_138/1 -> ObstacleDataA3/8  "ObstacleType"
  in_139/1 -> ObstacleDataA3/9  "reserved_1"
  in_140/1 -> ObstacleDataA3/10  "ObstacleStatus"
  in_141/1 -> ObstacleDataA3/11  "ObstacleBrakeLights"
  in_142/1 -> ObstacleDataA3/12  "reserved_2"
  in_143/1 -> ObstacleDataA3/13  "ObstacleValid"
  in_144/1 -> ObstacleDataA4/1  "ObstacleID"
  ObstacleDataA4/1 -> Mux/17  "ObstacleDataA4"
  in_145/1 -> ObstacleDataA4/2  "ObstaclePosX"
  in_146/1 -> ObstacleDataA4/3  "reserved_4"
  in_147/1 -> ObstacleDataA4/4  "ObstaclePosY"
  in_148/1 -> ObstacleDataA4/5  "BlinkerInfo"
  in_149/1 -> ObstacleDataA4/6  "Move_in_and_Out"
  in_150/1 -> ObstacleDataA4/7  "ObstacleVelX"
  in_151/1 -> ObstacleDataA4/8  "ObstacleType"
  in_152/1 -> ObstacleDataA4/9  "reserved_1"
  in_153/1 -> ObstacleDataA4/10  "ObstacleStatus"
  in_154/1 -> ObstacleDataA4/11  "ObstacleBrakeLights"
  in_155/1 -> ObstacleDataA4/12  "reserved_2"
  in_156/1 -> ObstacleDataA4/13  "ObstacleValid"
  in_157/1 -> ObstacleDataA5/1  "ObstacleID"
  ObstacleDataA5/1 -> Mux/18  "ObstacleDataA5"
  in_158/1 -> ObstacleDataA5/2  "ObstaclePosX"
  in_159/1 -> ObstacleDataA5/3  "reserved_4"
  in_160/1 -> ObstacleDataA5/4  "ObstaclePosY"
  in_161/1 -> ObstacleDataA5/5  "BlinkerInfo"
  in_162/1 -> ObstacleDataA5/6  "Move_in_and_Out"
  in_163/1 -> ObstacleDataA5/7  "ObstacleVelX"
  in_164/1 -> ObstacleDataA5/8  "ObstacleType"
  in_165/1 -> ObstacleDataA5/9  "reserved_1"
  in_166/1 -> ObstacleDataA5/10  "ObstacleStatus"
  in_167/1 -> ObstacleDataA5/11  "ObstacleBrakeLights"
  in_168/1 -> ObstacleDataA5/12  "reserved_2"
  in_169/1 -> ObstacleDataA5/13  "ObstacleValid"
  in_170/1 -> ObstacleDataA6/1  "ObstacleID"
  ObstacleDataA6/1 -> Mux/19  "ObstacleDataA6"
  in_171/1 -> ObstacleDataA6/2  "ObstaclePosX"
  in_172/1 -> ObstacleDataA6/3  "reserved_4"
  in_173/1 -> ObstacleDataA6/4  "ObstaclePosY"
  in_174/1 -> ObstacleDataA6/5  "BlinkerInfo"
  in_175/1 -> ObstacleDataA6/6  "Move_in_and_Out"
  in_176/1 -> ObstacleDataA6/7  "ObstacleVelX"
  in_177/1 -> ObstacleDataA6/8  "ObstacleType"
  in_178/1 -> ObstacleDataA6/9  "reserved_1"
  in_179/1 -> ObstacleDataA6/10  "ObstacleStatus"
  in_180/1 -> ObstacleDataA6/11  "ObstacleBrakeLights"
  in_181/1 -> ObstacleDataA6/12  "reserved_2"
  in_182/1 -> ObstacleDataA6/13  "ObstacleValid"
  in_183/1 -> ObstacleDataA7/1  "ObstacleID"
  ObstacleDataA7/1 -> Mux/20  "ObstacleDataA7"
  in_184/1 -> ObstacleDataA7/2  "ObstaclePosX"
  in_185/1 -> ObstacleDataA7/3  "reserved_4"
  in_186/1 -> ObstacleDataA7/4  "ObstaclePosY"
  in_187/1 -> ObstacleDataA7/5  "BlinkerInfo"
  in_188/1 -> ObstacleDataA7/6  "Move_in_and_Out"
  in_189/1 -> ObstacleDataA7/7  "ObstacleVelX"
  in_190/1 -> ObstacleDataA7/8  "ObstacleType"
  in_191/1 -> ObstacleDataA7/9  "reserved_1"
  in_192/1 -> ObstacleDataA7/10  "ObstacleStatus"
  in_193/1 -> ObstacleDataA7/11  "ObstacleBrakeLights"
  in_194/1 -> ObstacleDataA7/12  "reserved_2"
  in_195/1 -> ObstacleDataA7/13  "ObstacleValid"
  in_196/1 -> ObstacleDataA8/1  "ObstacleID"
  ObstacleDataA8/1 -> Mux/21  "ObstacleDataA8"
  in_197/1 -> ObstacleDataA8/2  "ObstaclePosX"
  in_198/1 -> ObstacleDataA8/3  "reserved_4"
  in_199/1 -> ObstacleDataA8/4  "ObstaclePosY"
  in_200/1 -> ObstacleDataA8/5  "BlinkerInfo"
  in_201/1 -> ObstacleDataA8/6  "Move_in_and_Out"
  in_202/1 -> ObstacleDataA8/7  "ObstacleVelX"
  in_203/1 -> ObstacleDataA8/8  "ObstacleType"
  in_204/1 -> ObstacleDataA8/9  "reserved_1"
  in_205/1 -> ObstacleDataA8/10  "ObstacleStatus"
  in_206/1 -> ObstacleDataA8/11  "ObstacleBrakeLights"
  in_207/1 -> ObstacleDataA8/12  "reserved_2"
  in_208/1 -> ObstacleDataA8/13  "ObstacleValid"
  in_209/1 -> ObstacleDataA9/1  "ObstacleID"
  ObstacleDataA9/1 -> Mux/22  "ObstacleDataA9"
  in_210/1 -> ObstacleDataA9/2  "ObstaclePosX"
  in_211/1 -> ObstacleDataA9/3  "reserved_4"
  in_212/1 -> ObstacleDataA9/4  "ObstaclePosY"
  in_213/1 -> ObstacleDataA9/5  "BlinkerInfo"
  in_214/1 -> ObstacleDataA9/6  "Move_in_and_Out"
  in_215/1 -> ObstacleDataA9/7  "ObstacleVelX"
  in_216/1 -> ObstacleDataA9/8  "ObstacleType"
  in_217/1 -> ObstacleDataA9/9  "reserved_1"
  in_218/1 -> ObstacleDataA9/10  "ObstacleStatus"
  in_219/1 -> ObstacleDataA9/11  "ObstacleBrakeLights"
  in_220/1 -> ObstacleDataA9/12  "reserved_2"
  in_221/1 -> ObstacleDataA9/13  "ObstacleValid"
  in_222/1 -> ObstacleDataB1/1  "ObstacleLength"
  ObstacleDataB1/1 -> Mux/23  "ObstacleDataB1"
  in_223/1 -> ObstacleDataB1/2  "ObstacleWidth"
  in_224/1 -> ObstacleDataB1/3  "ObstacleAge"
  in_225/1 -> ObstacleDataB1/4  "ObstacleLane"
  in_226/1 -> ObstacleDataB1/5  "CIPVFlag"
  in_227/1 -> ObstacleDataB1/6  "reserved_1"
  in_228/1 -> ObstacleDataB1/7  "RadarPosX"
  in_229/1 -> ObstacleDataB1/8  "RadarVelX"
  in_230/1 -> ObstacleDataB1/9  "RadarMatchConfidence"
  in_231/1 -> ObstacleDataB1/10  "reserved_1_b"
  in_232/1 -> ObstacleDataB1/11  "MatchedRadarID"
  in_233/1 -> ObstacleDataB1/12  "reserved_1_c"
  in_234/1 -> ObstacleDataB10/1  "ObstacleLength"
  ObstacleDataB10/1 -> Mux/24  "ObstacleDataB10"
  in_235/1 -> ObstacleDataB10/2  "ObstacleWidth"
  in_236/1 -> ObstacleDataB10/3  "ObstacleAge"
  in_237/1 -> ObstacleDataB10/4  "ObstacleLane"
  in_238/1 -> ObstacleDataB10/5  "CIPVFlag"
  in_239/1 -> ObstacleDataB10/6  "reserved_1"
  in_240/1 -> ObstacleDataB10/7  "RadarPosX"
  in_241/1 -> ObstacleDataB10/8  "RadarVelX"
  in_242/1 -> ObstacleDataB10/9  "RadarMatchConfidence"
  in_243/1 -> ObstacleDataB10/10  "reserved_1_b"
  in_244/1 -> ObstacleDataB10/11  "MatchedRadarID"
  in_245/1 -> ObstacleDataB10/12  "reserved_1_c"
  in_246/1 -> ObstacleDataB2/1  "ObstacleLength"
  ObstacleDataB2/1 -> Mux/25  "ObstacleDataB2"
  in_247/1 -> ObstacleDataB2/2  "ObstacleWidth"
  in_248/1 -> ObstacleDataB2/3  "ObstacleAge"
  in_249/1 -> ObstacleDataB2/4  "ObstacleLane"
  in_250/1 -> ObstacleDataB2/5  "CIPVFlag"
  in_251/1 -> ObstacleDataB2/6  "reserved_1"
  in_252/1 -> ObstacleDataB2/7  "RadarPosX"
  in_253/1 -> ObstacleDataB2/8  "RadarVelX"
  in_254/1 -> ObstacleDataB2/9  "RadarMatchConfidence"
  in_255/1 -> ObstacleDataB2/10  "reserved_1_b"
  in_256/1 -> ObstacleDataB2/11  "MatchedRadarID"
  in_257/1 -> ObstacleDataB2/12  "reserved_1_c"
  in_258/1 -> ObstacleDataB3/1  "ObstacleLength"
  ObstacleDataB3/1 -> Mux/26  "ObstacleDataB3"
  in_259/1 -> ObstacleDataB3/2  "ObstacleWidth"
  in_260/1 -> ObstacleDataB3/3  "ObstacleAge"
  in_261/1 -> ObstacleDataB3/4  "ObstacleLane"
  in_262/1 -> ObstacleDataB3/5  "CIPVFlag"
  in_263/1 -> ObstacleDataB3/6  "reserved_1"
  in_264/1 -> ObstacleDataB3/7  "RadarPosX"
  in_265/1 -> ObstacleDataB3/8  "RadarVelX"
  in_266/1 -> ObstacleDataB3/9  "RadarMatchConfidence"
  in_267/1 -> ObstacleDataB3/10  "reserved_1_b"
  in_268/1 -> ObstacleDataB3/11  "MatchedRadarID"
  in_269/1 -> ObstacleDataB3/12  "reserved_1_c"
  in_270/1 -> ObstacleDataB4/1  "ObstacleLength"
  ObstacleDataB4/1 -> Mux/27  "ObstacleDataB4"
  in_271/1 -> ObstacleDataB4/2  "ObstacleWidth"
  in_272/1 -> ObstacleDataB4/3  "ObstacleAge"
  in_273/1 -> ObstacleDataB4/4  "ObstacleLane"
  in_274/1 -> ObstacleDataB4/5  "CIPVFlag"
  in_275/1 -> ObstacleDataB4/6  "reserved_1"
  in_276/1 -> ObstacleDataB4/7  "RadarPosX"
  in_277/1 -> ObstacleDataB4/8  "RadarVelX"
  in_278/1 -> ObstacleDataB4/9  "RadarMatchConfidence"
  in_279/1 -> ObstacleDataB4/10  "reserved_1_b"
  in_280/1 -> ObstacleDataB4/11  "MatchedRadarID"
  in_281/1 -> ObstacleDataB4/12  "reserved_1_c"
  in_282/1 -> ObstacleDataB5/1  "ObstacleLength"
  ObstacleDataB5/1 -> Mux/28  "ObstacleDataB5"
  in_283/1 -> ObstacleDataB5/2  "ObstacleWidth"
  in_284/1 -> ObstacleDataB5/3  "ObstacleAge"
  in_285/1 -> ObstacleDataB5/4  "ObstacleLane"
  in_286/1 -> ObstacleDataB5/5  "CIPVFlag"
  in_287/1 -> ObstacleDataB5/6  "reserved_1"
  in_288/1 -> ObstacleDataB5/7  "RadarPosX"
  in_289/1 -> ObstacleDataB5/8  "RadarVelX"
  in_290/1 -> ObstacleDataB5/9  "RadarMatchConfidence"
  in_291/1 -> ObstacleDataB5/10  "reserved_1_b"
  in_292/1 -> ObstacleDataB5/11  "MatchedRadarID"
  in_293/1 -> ObstacleDataB5/12  "reserved_1_c"
  in_294/1 -> ObstacleDataB6/1  "ObstacleLength"
  ObstacleDataB6/1 -> Mux/29  "ObstacleDataB6"
  in_295/1 -> ObstacleDataB6/2  "ObstacleWidth"
  in_296/1 -> ObstacleDataB6/3  "ObstacleAge"
  in_297/1 -> ObstacleDataB6/4  "ObstacleLane"
  in_298/1 -> ObstacleDataB6/5  "CIPVFlag"
  in_299/1 -> ObstacleDataB6/6  "reserved_1"
  in_300/1 -> ObstacleDataB6/7  "RadarPosX"
  in_301/1 -> ObstacleDataB6/8  "RadarVelX"
  in_302/1 -> ObstacleDataB6/9  "RadarMatchConfidence"
  in_303/1 -> ObstacleDataB6/10  "reserved_1_b"
  in_304/1 -> ObstacleDataB6/11  "MatchedRadarID"
  in_305/1 -> ObstacleDataB6/12  "reserved_1_c"
  in_306/1 -> ObstacleDataB7/1  "ObstacleLength"
  ObstacleDataB7/1 -> Mux/30  "ObstacleDataB7"
  in_307/1 -> ObstacleDataB7/2  "ObstacleWidth"
  in_308/1 -> ObstacleDataB7/3  "ObstacleAge"
  in_309/1 -> ObstacleDataB7/4  "ObstacleLane"
  in_310/1 -> ObstacleDataB7/5  "CIPVFlag"
  in_311/1 -> ObstacleDataB7/6  "reserved_1"
  in_312/1 -> ObstacleDataB7/7  "RadarPosX"
  in_313/1 -> ObstacleDataB7/8  "RadarVelX"
  in_314/1 -> ObstacleDataB7/9  "RadarMatchConfidence"
  in_315/1 -> ObstacleDataB7/10  "reserved_1_b"
  in_316/1 -> ObstacleDataB7/11  "MatchedRadarID"
  in_317/1 -> ObstacleDataB7/12  "reserved_1_c"
  in_318/1 -> ObstacleDataB8/1  "ObstacleLength"
  ObstacleDataB8/1 -> Mux/31  "ObstacleDataB8"
  in_319/1 -> ObstacleDataB8/2  "ObstacleWidth"
  in_320/1 -> ObstacleDataB8/3  "ObstacleAge"
  in_321/1 -> ObstacleDataB8/4  "ObstacleLane"
  in_322/1 -> ObstacleDataB8/5  "CIPVFlag"
  in_323/1 -> ObstacleDataB8/6  "reserved_1"
  in_324/1 -> ObstacleDataB8/7  "RadarPosX"
  in_325/1 -> ObstacleDataB8/8  "RadarVelX"
  in_326/1 -> ObstacleDataB8/9  "RadarMatchConfidence"
  in_327/1 -> ObstacleDataB8/10  "reserved_1_b"
  in_328/1 -> ObstacleDataB8/11  "MatchedRadarID"
  in_329/1 -> ObstacleDataB8/12  "reserved_1_c"
  in_330/1 -> ObstacleDataB9/1  "ObstacleLength"
  ObstacleDataB9/1 -> Mux/32  "ObstacleDataB9"
  in_331/1 -> ObstacleDataB9/2  "ObstacleWidth"
  in_332/1 -> ObstacleDataB9/3  "ObstacleAge"
  in_333/1 -> ObstacleDataB9/4  "ObstacleLane"
  in_334/1 -> ObstacleDataB9/5  "CIPVFlag"
  in_335/1 -> ObstacleDataB9/6  "reserved_1"
  in_336/1 -> ObstacleDataB9/7  "RadarPosX"
  in_337/1 -> ObstacleDataB9/8  "RadarVelX"
  in_338/1 -> ObstacleDataB9/9  "RadarMatchConfidence"
  in_339/1 -> ObstacleDataB9/10  "reserved_1_b"
  in_340/1 -> ObstacleDataB9/11  "MatchedRadarID"
  in_341/1 -> ObstacleDataB9/12  "reserved_1_c"
  in_342/1 -> ObstacleDataC1/1  "ObstacleAngleRate"
  ObstacleDataC1/1 -> Mux/33  "ObstacleDataC1"
  in_343/1 -> ObstacleDataC1/2  "ObstacleVelY"
  in_344/1 -> ObstacleDataC1/3  "reserved_5"
  in_345/1 -> ObstacleDataC1/4  "Object_Accel_X"
  in_346/1 -> ObstacleDataC1/5  "reserved_2"
  in_347/1 -> ObstacleDataC1/6  "ObstacleReplaced"
  in_348/1 -> ObstacleDataC1/7  "reserved_3"
  in_349/1 -> ObstacleDataC1/8  "ObstacleAngle"
  in_350/1 -> ObstacleDataC10/1  "ObstacleAngleRate"
  ObstacleDataC10/1 -> Mux/34  "ObstacleDataC10"
  in_351/1 -> ObstacleDataC10/2  "ObstacleVelY"
  in_352/1 -> ObstacleDataC10/3  "reserved_5"
  in_353/1 -> ObstacleDataC10/4  "Object_Accel_X"
  in_354/1 -> ObstacleDataC10/5  "reserved_2"
  in_355/1 -> ObstacleDataC10/6  "ObstacleReplaced"
  in_356/1 -> ObstacleDataC10/7  "reserved_3"
  in_357/1 -> ObstacleDataC10/8  "ObstacleAngle"
  in_358/1 -> ObstacleDataC2/1  "ObstacleAngleRate"
  ObstacleDataC2/1 -> Mux/35  "ObstacleDataC2"
  in_359/1 -> ObstacleDataC2/2  "ObstacleVelY"
  in_360/1 -> ObstacleDataC2/3  "reserved_5"
  in_361/1 -> ObstacleDataC2/4  "Object_Accel_X"
  in_362/1 -> ObstacleDataC2/5  "reserved_2"
  in_363/1 -> ObstacleDataC2/6  "ObstacleReplaced"
  in_364/1 -> ObstacleDataC2/7  "reserved_3"
  in_365/1 -> ObstacleDataC2/8  "ObstacleAngle"
  in_366/1 -> ObstacleDataC3/1  "ObstacleAngleRate"
  ObstacleDataC3/1 -> Mux/36  "ObstacleDataC3"
  in_367/1 -> ObstacleDataC3/2  "ObstacleVelY"
  in_368/1 -> ObstacleDataC3/3  "reserved_5"
  in_369/1 -> ObstacleDataC3/4  "Object_Accel_X"
  in_370/1 -> ObstacleDataC3/5  "reserved_2"
  in_371/1 -> ObstacleDataC3/6  "ObstacleReplaced"
  in_372/1 -> ObstacleDataC3/7  "reserved_3"
  in_373/1 -> ObstacleDataC3/8  "ObstacleAngle"
  in_374/1 -> ObstacleDataC4/1  "ObstacleAngleRate"
  ObstacleDataC4/1 -> Mux/37  "ObstacleDataC4"
  in_375/1 -> ObstacleDataC4/2  "ObstacleVelY"
  in_376/1 -> ObstacleDataC4/3  "reserved_5"
  in_377/1 -> ObstacleDataC4/4  "Object_Accel_X"
  in_378/1 -> ObstacleDataC4/5  "reserved_2"
  in_379/1 -> ObstacleDataC4/6  "ObstacleReplaced"
  in_380/1 -> ObstacleDataC4/7  "reserved_3"
  in_381/1 -> ObstacleDataC4/8  "ObstacleAngle"
  in_382/1 -> ObstacleDataC5/1  "ObstacleAngleRate"
  ObstacleDataC5/1 -> Mux/38  "ObstacleDataC5"
  in_383/1 -> ObstacleDataC5/2  "ObstacleVelY"
  in_384/1 -> ObstacleDataC5/3  "reserved_5"
  in_385/1 -> ObstacleDataC5/4  "Object_Accel_X"
  in_386/1 -> ObstacleDataC5/5  "reserved_2"
  in_387/1 -> ObstacleDataC5/6  "ObstacleReplaced"
  in_388/1 -> ObstacleDataC5/7  "reserved_3"
  in_389/1 -> ObstacleDataC5/8  "ObstacleAngle"
  in_390/1 -> ObstacleDataC6/1  "ObstacleAngleRate"
  ObstacleDataC6/1 -> Mux/39  "ObstacleDataC6"
  in_391/1 -> ObstacleDataC6/2  "ObstacleVelY"
  in_392/1 -> ObstacleDataC6/3  "reserved_5"
  in_393/1 -> ObstacleDataC6/4  "Object_Accel_X"
  in_394/1 -> ObstacleDataC6/5  "reserved_2"
  in_395/1 -> ObstacleDataC6/6  "ObstacleReplaced"
  in_396/1 -> ObstacleDataC6/7  "reserved_3"
  in_397/1 -> ObstacleDataC6/8  "ObstacleAngle"
  in_398/1 -> ObstacleDataC7/1  "ObstacleAngleRate"
  ObstacleDataC7/1 -> Mux/40  "ObstacleDataC7"
  in_399/1 -> ObstacleDataC7/2  "ObstacleVelY"
  in_400/1 -> ObstacleDataC7/3  "reserved_5"
  in_401/1 -> ObstacleDataC7/4  "Object_Accel_X"
  in_402/1 -> ObstacleDataC7/5  "reserved_2"
  in_403/1 -> ObstacleDataC7/6  "ObstacleReplaced"
  in_404/1 -> ObstacleDataC7/7  "reserved_3"
  in_405/1 -> ObstacleDataC7/8  "ObstacleAngle"
  in_406/1 -> ObstacleDataC8/1  "ObstacleAngleRate"
  ObstacleDataC8/1 -> Mux/41  "ObstacleDataC8"
  in_407/1 -> ObstacleDataC8/2  "ObstacleVelY"
  in_408/1 -> ObstacleDataC8/3  "reserved_5"
  in_409/1 -> ObstacleDataC8/4  "Object_Accel_X"
  in_410/1 -> ObstacleDataC8/5  "reserved_2"
  in_411/1 -> ObstacleDataC8/6  "ObstacleReplaced"
  in_412/1 -> ObstacleDataC8/7  "reserved_3"
  in_413/1 -> ObstacleDataC8/8  "ObstacleAngle"
  in_414/1 -> ObstacleDataC9/1  "ObstacleAngleRate"
  ObstacleDataC9/1 -> Mux/42  "ObstacleDataC9"
  in_415/1 -> ObstacleDataC9/2  "ObstacleVelY"
  in_416/1 -> ObstacleDataC9/3  "reserved_5"
  in_417/1 -> ObstacleDataC9/4  "Object_Accel_X"
  in_418/1 -> ObstacleDataC9/5  "reserved_2"
  in_419/1 -> ObstacleDataC9/6  "ObstacleReplaced"
  in_420/1 -> ObstacleDataC9/7  "reserved_3"
  in_421/1 -> ObstacleDataC9/8  "ObstacleAngle"
  in_422/1 -> ObstacleStatusA/1  "NumObstacles"
  ObstacleStatusA/1 -> Mux/43  "ObstacleStatusA"
  in_423/1 -> ObstacleStatusA/2  "Timestamp"
  in_424/1 -> ObstacleStatusA/3  "ApplicationVersion_minor"
  in_425/1 -> ObstacleStatusA/4  "ApplicationVersion_rc"
  in_426/1 -> ObstacleStatusA/5  "ProtocolVersion"
  in_427/1 -> ObstacleStatusA/6  "Go"
  in_428/1 -> ObstacleStatusA/7  "Close_Car"
  in_429/1 -> ObstacleStatusA/8  "RightCloseRangeCutIn"
  in_430/1 -> ObstacleStatusA/9  "LeftCloseRangeCutIn"
  in_431/1 -> ObstacleStatusA/10  "Failsafe"
  in_432/1 -> ObstacleStatusA/11  "reserved_3"
  in_433/1 -> ObstacleStatusB/1  "timeStamp"
  ObstacleStatusB/1 -> Mux/44  "ObstacleStatusB"
  in_434/1 -> ObstacleStatusB/2  "frameIndex"
  in_435/1 -> ObstacleStatusC/1  "grabIndex"
  ObstacleStatusC/1 -> Mux/45  "ObstacleStatusC"
  in_436/1 -> ObstacleStatusC/2  "pedalConfGenObjDistFromBumper"
  in_437/1 -> ObstacleStatusC/3  "pedalConfusionGeneralObjTTC"
  in_438/1 -> ObstacleStatusC/4  "reserved_6"
  in_439/1 -> Road_Information/1  "Construction_Area"
  Road_Information/1 -> Mux/46  "Road_Information"
  in_440/1 -> Road_Information/2  "Road_Type"
  in_441/1 -> Road_Information/3  "Highway_Exit_Right"
  in_442/1 -> Road_Information/4  "Highway_Exit_Left"
  in_443/1 -> Road_Information/5  "Probability_Of_Left_Lane"
  in_444/1 -> Road_Information/6  "Probability_Of_Right_Lane"
  in_445/1 -> Road_Information/7  "Driving_Speed_Left_Lane"
  in_446/1 -> Road_Information/8  "Driving_Speed_Right_Lane"
  in_447/1 -> Road_Information/9  "protocol_version"
  in_448/1 -> RTICANMMCaptureMessage_1/1  "Status"
  RTICANMMCaptureMessage_1/1 -> Mux/47  "RTICANMMCaptureMessage_1"
  in_449/1 -> RTICANMMCaptureMessage_1/2  "Time"
  in_450/1 -> RTICANMMCaptureMessage_1/3  "ID"
  in_451/1 -> RTICANMMCaptureMessage_1/4  "MessageIDFormat"
  in_452/1 -> RTICANMMCaptureMessage_1/5  "Length"
  in_453/1 -> RTICANMMCaptureMessage_1/6  "RAW_Byte_1"
  in_454/1 -> RTICANMMCaptureMessage_1/7  "RAW_Byte_2"
  in_455/1 -> RTICANMMCaptureMessage_1/8  "RAW_Byte_3"
  in_456/1 -> RTICANMMCaptureMessage_1/9  "RAW_Byte_4"
  in_457/1 -> RTICANMMCaptureMessage_1/10  "RAW_Byte_5"
  in_458/1 -> RTICANMMCaptureMessage_1/11  "RAW_Byte_6"
  in_459/1 -> RTICANMMCaptureMessage_1/12  "RAW_Byte_7"
  in_460/1 -> RTICANMMCaptureMessage_1/13  "RAW_Byte_8"
  in_461/1 -> RTICANMMCaptureMessage_2/1  "Status"
  RTICANMMCaptureMessage_2/1 -> Mux/48  "RTICANMMCaptureMessage_2"
  in_462/1 -> RTICANMMCaptureMessage_2/2  "Time"
  in_463/1 -> RTICANMMCaptureMessage_2/3  "ID"
  in_464/1 -> RTICANMMCaptureMessage_2/4  "MessageIDFormat"
  in_465/1 -> RTICANMMCaptureMessage_2/5  "Length"
  in_466/1 -> RTICANMMCaptureMessage_2/6  "RAW_Byte_1"
  in_467/1 -> RTICANMMCaptureMessage_2/7  "RAW_Byte_2"
  in_468/1 -> RTICANMMCaptureMessage_2/8  "RAW_Byte_3"
  in_469/1 -> RTICANMMCaptureMessage_2/9  "RAW_Byte_4"
  in_470/1 -> RTICANMMCaptureMessage_2/10  "RAW_Byte_5"
  in_471/1 -> RTICANMMCaptureMessage_2/11  "RAW_Byte_6"
  in_472/1 -> RTICANMMCaptureMessage_2/12  "RAW_Byte_7"
  in_473/1 -> RTICANMMCaptureMessage_2/13  "RAW_Byte_8"
  in_474/1 -> RTICANMMCaptureMessage_3/1  "Status"
  RTICANMMCaptureMessage_3/1 -> Mux/49  "RTICANMMCaptureMessage_3"
  in_475/1 -> RTICANMMCaptureMessage_3/2  "Time"
  in_476/1 -> RTICANMMCaptureMessage_3/3  "ID"
  in_477/1 -> RTICANMMCaptureMessage_3/4  "MessageIDFormat"
  in_478/1 -> RTICANMMCaptureMessage_3/5  "Length"
  in_479/1 -> RTICANMMCaptureMessage_3/6  "RAW_Byte_1"
  in_480/1 -> RTICANMMCaptureMessage_3/7  "RAW_Byte_2"
  in_481/1 -> RTICANMMCaptureMessage_3/8  "RAW_Byte_3"
  in_482/1 -> RTICANMMCaptureMessage_3/9  "RAW_Byte_4"
  in_483/1 -> RTICANMMCaptureMessage_3/10  "RAW_Byte_5"
  in_484/1 -> RTICANMMCaptureMessage_3/11  "RAW_Byte_6"
  in_485/1 -> RTICANMMCaptureMessage_3/12  "RAW_Byte_7"
  in_486/1 -> RTICANMMCaptureMessage_3/13  "RAW_Byte_8"
  in_487/1 -> RTICANMMCaptureMessage_4/1  "Status"
  RTICANMMCaptureMessage_4/1 -> Mux/50  "RTICANMMCaptureMessage_4"
  in_488/1 -> RTICANMMCaptureMessage_4/2  "Time"
  in_489/1 -> RTICANMMCaptureMessage_4/3  "ID"
  in_490/1 -> RTICANMMCaptureMessage_4/4  "MessageIDFormat"
  in_491/1 -> RTICANMMCaptureMessage_4/5  "Length"
  in_492/1 -> RTICANMMCaptureMessage_4/6  "RAW_Byte_1"
  in_493/1 -> RTICANMMCaptureMessage_4/7  "RAW_Byte_2"
  in_494/1 -> RTICANMMCaptureMessage_4/8  "RAW_Byte_3"
  in_495/1 -> RTICANMMCaptureMessage_4/9  "RAW_Byte_4"
  in_496/1 -> RTICANMMCaptureMessage_4/10  "RAW_Byte_5"
  in_497/1 -> RTICANMMCaptureMessage_4/11  "RAW_Byte_6"
  in_498/1 -> RTICANMMCaptureMessage_4/12  "RAW_Byte_7"
  in_499/1 -> RTICANMMCaptureMessage_4/13  "RAW_Byte_8"
  in_500/1 -> RTICANMMCaptureMessage_5/1  "Status"
  RTICANMMCaptureMessage_5/1 -> Mux/51  "RTICANMMCaptureMessage_5"
  in_501/1 -> RTICANMMCaptureMessage_5/2  "Time"
  in_502/1 -> RTICANMMCaptureMessage_5/3  "ID"
  in_503/1 -> RTICANMMCaptureMessage_5/4  "MessageIDFormat"
  in_504/1 -> RTICANMMCaptureMessage_5/5  "Length"
  in_505/1 -> RTICANMMCaptureMessage_5/6  "RAW_Byte_1"
  in_506/1 -> RTICANMMCaptureMessage_5/7  "RAW_Byte_2"
  in_507/1 -> RTICANMMCaptureMessage_5/8  "RAW_Byte_3"
  in_508/1 -> RTICANMMCaptureMessage_5/9  "RAW_Byte_4"
  in_509/1 -> RTICANMMCaptureMessage_5/10  "RAW_Byte_5"
  in_510/1 -> RTICANMMCaptureMessage_5/11  "RAW_Byte_6"
  in_511/1 -> RTICANMMCaptureMessage_5/12  "RAW_Byte_7"
  in_512/1 -> RTICANMMCaptureMessage_5/13  "RAW_Byte_8"
  in_513/1 -> RTICANMMCaptureMessage_6/1  "Status"
  RTICANMMCaptureMessage_6/1 -> Mux/52  "RTICANMMCaptureMessage_6"
  in_514/1 -> RTICANMMCaptureMessage_6/2  "Time"
  in_515/1 -> RTICANMMCaptureMessage_6/3  "ID"
  in_516/1 -> RTICANMMCaptureMessage_6/4  "MessageIDFormat"
  in_517/1 -> RTICANMMCaptureMessage_6/5  "Length"
  in_518/1 -> RTICANMMCaptureMessage_6/6  "RAW_Byte_1"
  in_519/1 -> RTICANMMCaptureMessage_6/7  "RAW_Byte_2"
  in_520/1 -> RTICANMMCaptureMessage_6/8  "RAW_Byte_3"
  in_521/1 -> RTICANMMCaptureMessage_6/9  "RAW_Byte_4"
  in_522/1 -> RTICANMMCaptureMessage_6/10  "RAW_Byte_5"
  in_523/1 -> RTICANMMCaptureMessage_6/11  "RAW_Byte_6"
  in_524/1 -> RTICANMMCaptureMessage_6/12  "RAW_Byte_7"
  in_525/1 -> RTICANMMCaptureMessage_6/13  "RAW_Byte_8"
  in_526/1 -> RTICANMMCaptureMessage_7/1  "Status"
  RTICANMMCaptureMessage_7/1 -> Mux/53  "RTICANMMCaptureMessage_7"
  in_527/1 -> RTICANMMCaptureMessage_7/2  "Time"
  in_528/1 -> RTICANMMCaptureMessage_7/3  "ID"
  in_529/1 -> RTICANMMCaptureMessage_7/4  "MessageIDFormat"
  in_530/1 -> RTICANMMCaptureMessage_7/5  "Length"
  in_531/1 -> RTICANMMCaptureMessage_7/6  "RAW_Byte_1"
  in_532/1 -> RTICANMMCaptureMessage_7/7  "RAW_Byte_2"
  in_533/1 -> RTICANMMCaptureMessage_7/8  "RAW_Byte_3"
  in_534/1 -> RTICANMMCaptureMessage_7/9  "RAW_Byte_4"
  in_535/1 -> RTICANMMCaptureMessage_7/10  "RAW_Byte_5"
  in_536/1 -> RTICANMMCaptureMessage_7/11  "RAW_Byte_6"
  in_537/1 -> RTICANMMCaptureMessage_7/12  "RAW_Byte_7"
  in_538/1 -> RTICANMMCaptureMessage_7/13  "RAW_Byte_8"
  in_539/1 -> RTICANMMCaptureMessage_8/1  "Status"
  RTICANMMCaptureMessage_8/1 -> Mux/54  "RTICANMMCaptureMessage_8"
  in_540/1 -> RTICANMMCaptureMessage_8/2  "Time"
  in_541/1 -> RTICANMMCaptureMessage_8/3  "ID"
  in_542/1 -> RTICANMMCaptureMessage_8/4  "MessageIDFormat"
  in_543/1 -> RTICANMMCaptureMessage_8/5  "Length"
  in_544/1 -> RTICANMMCaptureMessage_8/6  "RAW_Byte_1"
  in_545/1 -> RTICANMMCaptureMessage_8/7  "RAW_Byte_2"
  in_546/1 -> RTICANMMCaptureMessage_8/8  "RAW_Byte_3"
  in_547/1 -> RTICANMMCaptureMessage_8/9  "RAW_Byte_4"
  in_548/1 -> RTICANMMCaptureMessage_8/10  "RAW_Byte_5"
  in_549/1 -> RTICANMMCaptureMessage_8/11  "RAW_Byte_6"
  in_550/1 -> RTICANMMCaptureMessage_8/12  "RAW_Byte_7"
  in_551/1 -> RTICANMMCaptureMessage_8/13  "RAW_Byte_8"
  in_552/1 -> RTICANMMCaptureMessage_9/1  "Status"
  RTICANMMCaptureMessage_9/1 -> Mux/55  "RTICANMMCaptureMessage_9"
  in_553/1 -> RTICANMMCaptureMessage_9/2  "Time"
  in_554/1 -> RTICANMMCaptureMessage_9/3  "ID"
  in_555/1 -> RTICANMMCaptureMessage_9/4  "MessageIDFormat"
  in_556/1 -> RTICANMMCaptureMessage_9/5  "Length"
  in_557/1 -> RTICANMMCaptureMessage_9/6  "RAW_Byte_1"
  in_558/1 -> RTICANMMCaptureMessage_9/7  "RAW_Byte_2"
  in_559/1 -> RTICANMMCaptureMessage_9/8  "RAW_Byte_3"
  in_560/1 -> RTICANMMCaptureMessage_9/9  "RAW_Byte_4"
  in_561/1 -> RTICANMMCaptureMessage_9/10  "RAW_Byte_5"
  in_562/1 -> RTICANMMCaptureMessage_9/11  "RAW_Byte_6"
  in_563/1 -> RTICANMMCaptureMessage_9/12  "RAW_Byte_7"
  in_564/1 -> RTICANMMCaptureMessage_9/13  "RAW_Byte_8"
  in_565/1 -> RTICANMMCaptureMessage_10/1  "Status"
  RTICANMMCaptureMessage_10/1 -> Mux/56  "RTICANMMCaptureMessage_10"
  in_566/1 -> RTICANMMCaptureMessage_10/2  "Time"
  in_567/1 -> RTICANMMCaptureMessage_10/3  "ID"
  in_568/1 -> RTICANMMCaptureMessage_10/4  "MessageIDFormat"
  in_569/1 -> RTICANMMCaptureMessage_10/5  "Length"
  in_570/1 -> RTICANMMCaptureMessage_10/6  "RAW_Byte_1"
  in_571/1 -> RTICANMMCaptureMessage_10/7  "RAW_Byte_2"
  in_572/1 -> RTICANMMCaptureMessage_10/8  "RAW_Byte_3"
  in_573/1 -> RTICANMMCaptureMessage_10/9  "RAW_Byte_4"
  in_574/1 -> RTICANMMCaptureMessage_10/10  "RAW_Byte_5"
  in_575/1 -> RTICANMMCaptureMessage_10/11  "RAW_Byte_6"
  in_576/1 -> RTICANMMCaptureMessage_10/12  "RAW_Byte_7"
  in_577/1 -> RTICANMMCaptureMessage_10/13  "RAW_Byte_8"
  in_578/1 -> RTICANMMCaptureMessage_11/1  "Status"
  RTICANMMCaptureMessage_11/1 -> Mux/57  "RTICANMMCaptureMessage_11"
  in_579/1 -> RTICANMMCaptureMessage_11/2  "Time"
  in_580/1 -> RTICANMMCaptureMessage_11/3  "ID"
  in_581/1 -> RTICANMMCaptureMessage_11/4  "MessageIDFormat"
  in_582/1 -> RTICANMMCaptureMessage_11/5  "Length"
  in_583/1 -> RTICANMMCaptureMessage_11/6  "RAW_Byte_1"
  in_584/1 -> RTICANMMCaptureMessage_11/7  "RAW_Byte_2"
  in_585/1 -> RTICANMMCaptureMessage_11/8  "RAW_Byte_3"
  in_586/1 -> RTICANMMCaptureMessage_11/9  "RAW_Byte_4"
  in_587/1 -> RTICANMMCaptureMessage_11/10  "RAW_Byte_5"
  in_588/1 -> RTICANMMCaptureMessage_11/11  "RAW_Byte_6"
  in_589/1 -> RTICANMMCaptureMessage_11/12  "RAW_Byte_7"
  in_590/1 -> RTICANMMCaptureMessage_11/13  "RAW_Byte_8"
  in_591/1 -> RTICANMMCaptureMessage_12/1  "Status"
  RTICANMMCaptureMessage_12/1 -> Mux/58  "RTICANMMCaptureMessage_12"
  in_592/1 -> RTICANMMCaptureMessage_12/2  "Time"
  in_593/1 -> RTICANMMCaptureMessage_12/3  "ID"
  in_594/1 -> RTICANMMCaptureMessage_12/4  "MessageIDFormat"
  in_595/1 -> RTICANMMCaptureMessage_12/5  "Length"
  in_596/1 -> RTICANMMCaptureMessage_12/6  "RAW_Byte_1"
  in_597/1 -> RTICANMMCaptureMessage_12/7  "RAW_Byte_2"
  in_598/1 -> RTICANMMCaptureMessage_12/8  "RAW_Byte_3"
  in_599/1 -> RTICANMMCaptureMessage_12/9  "RAW_Byte_4"
  in_600/1 -> RTICANMMCaptureMessage_12/10  "RAW_Byte_5"
  in_601/1 -> RTICANMMCaptureMessage_12/11  "RAW_Byte_6"
  in_602/1 -> RTICANMMCaptureMessage_12/12  "RAW_Byte_7"
  in_603/1 -> RTICANMMCaptureMessage_12/13  "RAW_Byte_8"
  in_604/1 -> RTICANMMCaptureMessage_13/1  "Status"
  RTICANMMCaptureMessage_13/1 -> Mux/59  "RTICANMMCaptureMessage_13"
  in_605/1 -> RTICANMMCaptureMessage_13/2  "Time"
  in_606/1 -> RTICANMMCaptureMessage_13/3  "ID"
  in_607/1 -> RTICANMMCaptureMessage_13/4  "MessageIDFormat"
  in_608/1 -> RTICANMMCaptureMessage_13/5  "Length"
  in_609/1 -> RTICANMMCaptureMessage_13/6  "RAW_Byte_1"
  in_610/1 -> RTICANMMCaptureMessage_13/7  "RAW_Byte_2"
  in_611/1 -> RTICANMMCaptureMessage_13/8  "RAW_Byte_3"
  in_612/1 -> RTICANMMCaptureMessage_13/9  "RAW_Byte_4"
  in_613/1 -> RTICANMMCaptureMessage_13/10  "RAW_Byte_5"
  in_614/1 -> RTICANMMCaptureMessage_13/11  "RAW_Byte_6"
  in_615/1 -> RTICANMMCaptureMessage_13/12  "RAW_Byte_7"
  in_616/1 -> RTICANMMCaptureMessage_13/13  "RAW_Byte_8"
  in_617/1 -> RTICANMMCaptureMessage_14/1  "Status"
  RTICANMMCaptureMessage_14/1 -> Mux/60  "RTICANMMCaptureMessage_14"
  in_618/1 -> RTICANMMCaptureMessage_14/2  "Time"
  in_619/1 -> RTICANMMCaptureMessage_14/3  "ID"
  in_620/1 -> RTICANMMCaptureMessage_14/4  "MessageIDFormat"
  in_621/1 -> RTICANMMCaptureMessage_14/5  "Length"
  in_622/1 -> RTICANMMCaptureMessage_14/6  "RAW_Byte_1"
  in_623/1 -> RTICANMMCaptureMessage_14/7  "RAW_Byte_2"
  in_624/1 -> RTICANMMCaptureMessage_14/8  "RAW_Byte_3"
  in_625/1 -> RTICANMMCaptureMessage_14/9  "RAW_Byte_4"
  in_626/1 -> RTICANMMCaptureMessage_14/10  "RAW_Byte_5"
  in_627/1 -> RTICANMMCaptureMessage_14/11  "RAW_Byte_6"
  in_628/1 -> RTICANMMCaptureMessage_14/12  "RAW_Byte_7"
  in_629/1 -> RTICANMMCaptureMessage_14/13  "RAW_Byte_8"
  in_630/1 -> RTICANMMCaptureMessage_15/1  "Status"
  RTICANMMCaptureMessage_15/1 -> Mux/61  "RTICANMMCaptureMessage_15"
  in_631/1 -> RTICANMMCaptureMessage_15/2  "Time"
  in_632/1 -> RTICANMMCaptureMessage_15/3  "ID"
  in_633/1 -> RTICANMMCaptureMessage_15/4  "MessageIDFormat"
  in_634/1 -> RTICANMMCaptureMessage_15/5  "Length"
  in_635/1 -> RTICANMMCaptureMessage_15/6  "RAW_Byte_1"
  in_636/1 -> RTICANMMCaptureMessage_15/7  "RAW_Byte_2"
  in_637/1 -> RTICANMMCaptureMessage_15/8  "RAW_Byte_3"
  in_638/1 -> RTICANMMCaptureMessage_15/9  "RAW_Byte_4"
  in_639/1 -> RTICANMMCaptureMessage_15/10  "RAW_Byte_5"
  in_640/1 -> RTICANMMCaptureMessage_15/11  "RAW_Byte_6"
  in_641/1 -> RTICANMMCaptureMessage_15/12  "RAW_Byte_7"
  in_642/1 -> RTICANMMCaptureMessage_15/13  "RAW_Byte_8"
  in_643/1 -> RTICANMMCaptureMessage_16/1  "Status"
  RTICANMMCaptureMessage_16/1 -> Mux/62  "RTICANMMCaptureMessage_16"
  in_644/1 -> RTICANMMCaptureMessage_16/2  "Time"
  in_645/1 -> RTICANMMCaptureMessage_16/3  "ID"
  in_646/1 -> RTICANMMCaptureMessage_16/4  "MessageIDFormat"
  in_647/1 -> RTICANMMCaptureMessage_16/5  "Length"
  in_648/1 -> RTICANMMCaptureMessage_16/6  "RAW_Byte_1"
  in_649/1 -> RTICANMMCaptureMessage_16/7  "RAW_Byte_2"
  in_650/1 -> RTICANMMCaptureMessage_16/8  "RAW_Byte_3"
  in_651/1 -> RTICANMMCaptureMessage_16/9  "RAW_Byte_4"
  in_652/1 -> RTICANMMCaptureMessage_16/10  "RAW_Byte_5"
  in_653/1 -> RTICANMMCaptureMessage_16/11  "RAW_Byte_6"
  in_654/1 -> RTICANMMCaptureMessage_16/12  "RAW_Byte_7"
  in_655/1 -> RTICANMMCaptureMessage_16/13  "RAW_Byte_8"
  in_656/1 -> RTICANMMCaptureMessage_17/1  "Status"
  RTICANMMCaptureMessage_17/1 -> Mux/63  "RTICANMMCaptureMessage_17"
  in_657/1 -> RTICANMMCaptureMessage_17/2  "Time"
  in_658/1 -> RTICANMMCaptureMessage_17/3  "ID"
  in_659/1 -> RTICANMMCaptureMessage_17/4  "MessageIDFormat"
  in_660/1 -> RTICANMMCaptureMessage_17/5  "Length"
  in_661/1 -> RTICANMMCaptureMessage_17/6  "RAW_Byte_1"
  in_662/1 -> RTICANMMCaptureMessage_17/7  "RAW_Byte_2"
  in_663/1 -> RTICANMMCaptureMessage_17/8  "RAW_Byte_3"
  in_664/1 -> RTICANMMCaptureMessage_17/9  "RAW_Byte_4"
  in_665/1 -> RTICANMMCaptureMessage_17/10  "RAW_Byte_5"
  in_666/1 -> RTICANMMCaptureMessage_17/11  "RAW_Byte_6"
  in_667/1 -> RTICANMMCaptureMessage_17/12  "RAW_Byte_7"
  in_668/1 -> RTICANMMCaptureMessage_17/13  "RAW_Byte_8"
  in_669/1 -> RTICANMMCaptureMessage_18/1  "Status"
  RTICANMMCaptureMessage_18/1 -> Mux/64  "RTICANMMCaptureMessage_18"
  in_670/1 -> RTICANMMCaptureMessage_18/2  "Time"
  in_671/1 -> RTICANMMCaptureMessage_18/3  "ID"
  in_672/1 -> RTICANMMCaptureMessage_18/4  "MessageIDFormat"
  in_673/1 -> RTICANMMCaptureMessage_18/5  "Length"
  in_674/1 -> RTICANMMCaptureMessage_18/6  "RAW_Byte_1"
  in_675/1 -> RTICANMMCaptureMessage_18/7  "RAW_Byte_2"
  in_676/1 -> RTICANMMCaptureMessage_18/8  "RAW_Byte_3"
  in_677/1 -> RTICANMMCaptureMessage_18/9  "RAW_Byte_4"
  in_678/1 -> RTICANMMCaptureMessage_18/10  "RAW_Byte_5"
  in_679/1 -> RTICANMMCaptureMessage_18/11  "RAW_Byte_6"
  in_680/1 -> RTICANMMCaptureMessage_18/12  "RAW_Byte_7"
  in_681/1 -> RTICANMMCaptureMessage_18/13  "RAW_Byte_8"
  in_682/1 -> RTICANMMCaptureMessage_19/1  "Status"
  RTICANMMCaptureMessage_19/1 -> Mux/65  "RTICANMMCaptureMessage_19"
  in_683/1 -> RTICANMMCaptureMessage_19/2  "Time"
  in_684/1 -> RTICANMMCaptureMessage_19/3  "ID"
  in_685/1 -> RTICANMMCaptureMessage_19/4  "MessageIDFormat"
  in_686/1 -> RTICANMMCaptureMessage_19/5  "Length"
  in_687/1 -> RTICANMMCaptureMessage_19/6  "RAW_Byte_1"
  in_688/1 -> RTICANMMCaptureMessage_19/7  "RAW_Byte_2"
  in_689/1 -> RTICANMMCaptureMessage_19/8  "RAW_Byte_3"
  in_690/1 -> RTICANMMCaptureMessage_19/9  "RAW_Byte_4"
  in_691/1 -> RTICANMMCaptureMessage_19/10  "RAW_Byte_5"
  in_692/1 -> RTICANMMCaptureMessage_19/11  "RAW_Byte_6"
  in_693/1 -> RTICANMMCaptureMessage_19/12  "RAW_Byte_7"
  in_694/1 -> RTICANMMCaptureMessage_19/13  "RAW_Byte_8"
  in_695/1 -> RTICANMMCaptureMessage_20/1  "Status"
  RTICANMMCaptureMessage_20/1 -> Mux/66  "RTICANMMCaptureMessage_20"
  in_696/1 -> RTICANMMCaptureMessage_20/2  "Time"
  in_697/1 -> RTICANMMCaptureMessage_20/3  "ID"
  in_698/1 -> RTICANMMCaptureMessage_20/4  "MessageIDFormat"
  in_699/1 -> RTICANMMCaptureMessage_20/5  "Length"
  in_700/1 -> RTICANMMCaptureMessage_20/6  "RAW_Byte_1"
  in_701/1 -> RTICANMMCaptureMessage_20/7  "RAW_Byte_2"
  in_702/1 -> RTICANMMCaptureMessage_20/8  "RAW_Byte_3"
  in_703/1 -> RTICANMMCaptureMessage_20/9  "RAW_Byte_4"
  in_704/1 -> RTICANMMCaptureMessage_20/10  "RAW_Byte_5"
  in_705/1 -> RTICANMMCaptureMessage_20/11  "RAW_Byte_6"
  in_706/1 -> RTICANMMCaptureMessage_20/12  "RAW_Byte_7"
  in_707/1 -> RTICANMMCaptureMessage_20/13  "RAW_Byte_8"
  in_708/1 -> RTICANMMCaptureMessage_21/1  "Status"
  RTICANMMCaptureMessage_21/1 -> Mux/67  "RTICANMMCaptureMessage_21"
  in_709/1 -> RTICANMMCaptureMessage_21/2  "Time"
  in_710/1 -> RTICANMMCaptureMessage_21/3  "ID"
  in_711/1 -> RTICANMMCaptureMessage_21/4  "MessageIDFormat"
  in_712/1 -> RTICANMMCaptureMessage_21/5  "Length"
  in_713/1 -> RTICANMMCaptureMessage_21/6  "RAW_Byte_1"
  in_714/1 -> RTICANMMCaptureMessage_21/7  "RAW_Byte_2"
  in_715/1 -> RTICANMMCaptureMessage_21/8  "RAW_Byte_3"
  in_716/1 -> RTICANMMCaptureMessage_21/9  "RAW_Byte_4"
  in_717/1 -> RTICANMMCaptureMessage_21/10  "RAW_Byte_5"
  in_718/1 -> RTICANMMCaptureMessage_21/11  "RAW_Byte_6"
  in_719/1 -> RTICANMMCaptureMessage_21/12  "RAW_Byte_7"
  in_720/1 -> RTICANMMCaptureMessage_21/13  "RAW_Byte_8"
  in_721/1 -> RTICANMMCaptureMessage_22/1  "Status"
  RTICANMMCaptureMessage_22/1 -> Mux/68  "RTICANMMCaptureMessage_22"
  in_722/1 -> RTICANMMCaptureMessage_22/2  "Time"
  in_723/1 -> RTICANMMCaptureMessage_22/3  "ID"
  in_724/1 -> RTICANMMCaptureMessage_22/4  "MessageIDFormat"
  in_725/1 -> RTICANMMCaptureMessage_22/5  "Length"
  in_726/1 -> RTICANMMCaptureMessage_22/6  "RAW_Byte_1"
  in_727/1 -> RTICANMMCaptureMessage_22/7  "RAW_Byte_2"
  in_728/1 -> RTICANMMCaptureMessage_22/8  "RAW_Byte_3"
  in_729/1 -> RTICANMMCaptureMessage_22/9  "RAW_Byte_4"
  in_730/1 -> RTICANMMCaptureMessage_22/10  "RAW_Byte_5"
  in_731/1 -> RTICANMMCaptureMessage_22/11  "RAW_Byte_6"
  in_732/1 -> RTICANMMCaptureMessage_22/12  "RAW_Byte_7"
  in_733/1 -> RTICANMMCaptureMessage_22/13  "RAW_Byte_8"
  in_734/1 -> RTICANMMCaptureMessage_23/1  "Status"
  RTICANMMCaptureMessage_23/1 -> Mux/69  "RTICANMMCaptureMessage_23"
  in_735/1 -> RTICANMMCaptureMessage_23/2  "Time"
  in_736/1 -> RTICANMMCaptureMessage_23/3  "ID"
  in_737/1 -> RTICANMMCaptureMessage_23/4  "MessageIDFormat"
  in_738/1 -> RTICANMMCaptureMessage_23/5  "Length"
  in_739/1 -> RTICANMMCaptureMessage_23/6  "RAW_Byte_1"
  in_740/1 -> RTICANMMCaptureMessage_23/7  "RAW_Byte_2"
  in_741/1 -> RTICANMMCaptureMessage_23/8  "RAW_Byte_3"
  in_742/1 -> RTICANMMCaptureMessage_23/9  "RAW_Byte_4"
  in_743/1 -> RTICANMMCaptureMessage_23/10  "RAW_Byte_5"
  in_744/1 -> RTICANMMCaptureMessage_23/11  "RAW_Byte_6"
  in_745/1 -> RTICANMMCaptureMessage_23/12  "RAW_Byte_7"
  in_746/1 -> RTICANMMCaptureMessage_23/13  "RAW_Byte_8"
  in_747/1 -> RTICANMMCaptureMessage_24/1  "Status"
  RTICANMMCaptureMessage_24/1 -> Mux/70  "RTICANMMCaptureMessage_24"
  in_748/1 -> RTICANMMCaptureMessage_24/2  "Time"
  in_749/1 -> RTICANMMCaptureMessage_24/3  "ID"
  in_750/1 -> RTICANMMCaptureMessage_24/4  "MessageIDFormat"
  in_751/1 -> RTICANMMCaptureMessage_24/5  "Length"
  in_752/1 -> RTICANMMCaptureMessage_24/6  "RAW_Byte_1"
  in_753/1 -> RTICANMMCaptureMessage_24/7  "RAW_Byte_2"
  in_754/1 -> RTICANMMCaptureMessage_24/8  "RAW_Byte_3"
  in_755/1 -> RTICANMMCaptureMessage_24/9  "RAW_Byte_4"
  in_756/1 -> RTICANMMCaptureMessage_24/10  "RAW_Byte_5"
  in_757/1 -> RTICANMMCaptureMessage_24/11  "RAW_Byte_6"
  in_758/1 -> RTICANMMCaptureMessage_24/12  "RAW_Byte_7"
  in_759/1 -> RTICANMMCaptureMessage_24/13  "RAW_Byte_8"
  in_760/1 -> RTICANMMCaptureMessage_25/1  "Status"
  RTICANMMCaptureMessage_25/1 -> Mux/71  "RTICANMMCaptureMessage_25"
  in_761/1 -> RTICANMMCaptureMessage_25/2  "Time"
  in_762/1 -> RTICANMMCaptureMessage_25/3  "ID"
  in_763/1 -> RTICANMMCaptureMessage_25/4  "MessageIDFormat"
  in_764/1 -> RTICANMMCaptureMessage_25/5  "Length"
  in_765/1 -> RTICANMMCaptureMessage_25/6  "RAW_Byte_1"
  in_766/1 -> RTICANMMCaptureMessage_25/7  "RAW_Byte_2"
  in_767/1 -> RTICANMMCaptureMessage_25/8  "RAW_Byte_3"
  in_768/1 -> RTICANMMCaptureMessage_25/9  "RAW_Byte_4"
  in_769/1 -> RTICANMMCaptureMessage_25/10  "RAW_Byte_5"
  in_770/1 -> RTICANMMCaptureMessage_25/11  "RAW_Byte_6"
  in_771/1 -> RTICANMMCaptureMessage_25/12  "RAW_Byte_7"
  in_772/1 -> RTICANMMCaptureMessage_25/13  "RAW_Byte_8"
  Mux/1 -> out/1
